simulink model "StateMachine_v3"  (R2015a)
settings: Solver=ode1  StartTime=0.0  StopTime=Inf  FixedStep=0.001  RelTol=1e-3
PreLoadFcn:
  | LoadVar
PostLoadFcn:
  | , if any(exist('dsrtsu_mdlpostloadfcn', 'file') == [2, 3, 6]), try dsrtsu_mdlpostloadfcn('Execute', bdroot); catch fprintf('Error in PostLoadFcn (dsrtsu_mdlpostloadfcn) for model "%s":\n %s\n', bdroot, lasterr); end, end,
values from neighbouring files (symbols this model uses):
  AllowReset = 0    [LoadVar.m]
  Brake_Limits = [Brake_lowerlim1,Brake_upperlim1,Brake_lowerlim2,Brake_upperlim2]    [LoadVar.m]
  DcCLimGen = 0    [LoadVar.m]
  DcCLimMot = 20    [LoadVar.m]
  DcVLimGen = 400    [LoadVar.m]
  DcVLimMot = 280    [LoadVar.m]
  DifferentialFactor = 0.5    [LoadVar.m]
  MaxDisplacementSteeringRack = 21.08    [LoadVar.m]
  MaxSteeringAngle = 24.635    [LoadVar.m]
  MechPwrMaxGen = 3000    [LoadVar.m]
  MechPwrMaxMot = 3000    [LoadVar.m]
  PowerLim_W = 3000    [LoadVar.m]
  SpdSlewrate = 1000    [LoadVar.m]
  Steer_Limits = [Steer_lowerlim,Steer_upperlim,Steer_zero]    [LoadVar.m]
  Susp_Limits = [Susp_lowerlim1,Susp_upperlim1,Susp_lowerlim2,Susp_upperlim2,Susp_lowerlim3,Susp_upperlim3,Susp_lowerlim4,Susp_upperlim4]    [LoadVar.m]
  Throttle_Limits = [Throttle_lowerlim1,Throttle_upperlim1,Throttle_lowerlim2,Throttle_upperlim2]    [LoadVar.m]
  TrqSlewrate = 3    [LoadVar.m]
libraries: rtican x25, rti1401lib_adc_type4 x16, rti1401lib_dio_type3 x16, rtilib1401 x1
(part 3 of 7)

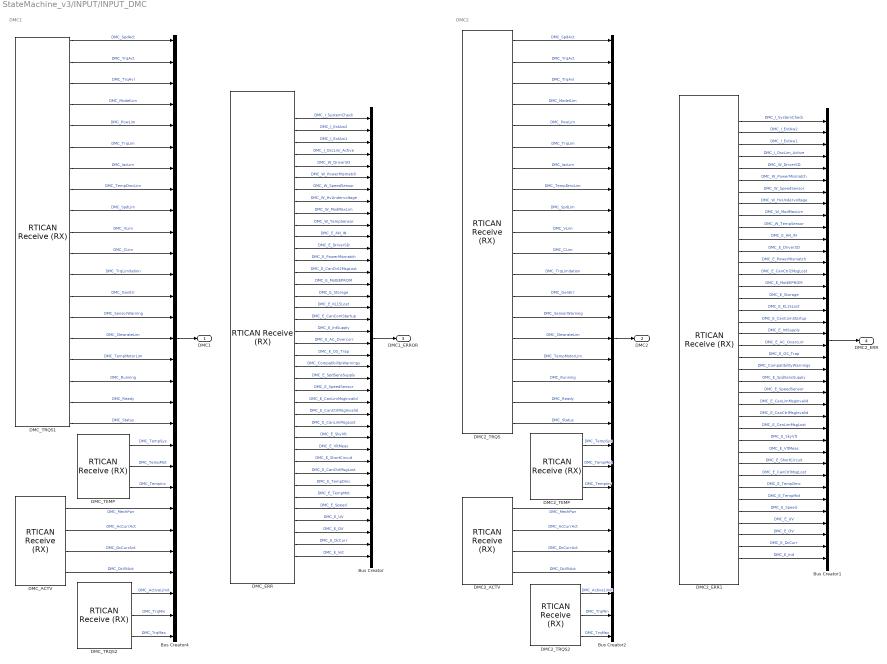
== system StateMachine_v3/INPUT/INPUT_DMC ==
  note: DMC2
  note: DMC1
  Bus Creator : BusCreator  Inputs=38
  Bus Creator1 : BusCreator  Inputs=38
  Bus Creator2 : BusCreator  Inputs=29
  Bus Creator4 : BusCreator  Inputs=29
  DMC2_ACTV : rtican/RTICAN Receive (RX)   Reserved1=[]  Reserved2=[]  Reserved3=[]  Reserved4=[]  SfcnMessage=[]  Msg_Struct=[]  BoardTypeNo=[]  BoardNo=[]  ChannelNo=[]  Parameters=[]  DialogFcn=[]  UnitName=[]  Revision=[]  UnitValues=[]  DSProperties=struct('RTI',struct('Version',uint32(5),'BlockType',struct('isSLSource',uint8(1),'isSLSink',uint8(1),'isHWSource',uint8(0),'isHWSink',uint8(0),'isSetup',uint8(0),'isInline',uint8(1),'isNonInline',uint8(0),'isInterrupt',uint8(0),'isChannelwise',uint8(0)),'IOBoardType','RTICAN','UnitType','MESSAGE','Identifier','RX','DialogType','MSVC','BlockSet','RTICAN','SlaveProcessor','CAN'))  RTIBlockInterface=struct('OutputPortsWidth',int32([1 1 1 1]),'OutputPortsActive',[1 1 1 1],'OutputPortsName',{{'DMC_MechPwr','DMC_AcCurrAct','DMC_DcCurrAct','DMC_DcVltAct'}},'OutputPortsDataType',{{'SS_DOUBLE','SS_DOUBLE','SS_DOUBLE','SS_DOUBLE'}},'OutputPortsLabel',{{'DMC_MechPwr','DMC_AcCurrAct','DMC_DcCurrAct','DMC_DcVltAct'}},'OutputPortsLabelMode','ON','InputPortsWidth',int32(0),'InputPortsActive',0,'DialogFcn','rtican_message_interface_gui','BlockDisplay',{{'','center'}},'IconTransparency','on','ParameterTunableNames',{{}},'InitLevel',3,'BlockName',struct('Token',{{'DMC2_ACTV'}}),'SampleTime',{{-1}},'TriggerPort',{{'none'}},'EnablePort',{{'none'}})  RTIBlockParameters=struct('BoardTypeNo',{{1,'OFF',[]}},'BoardNo',{{2,'ON',[1 16]}},'ChannelNo',{{1,'ON',[1 2]}},'Parameters',{{struct('DataFileSupport',struct('DataFileSelectedMaster',1,'DataFileSelectedLocal',0,'DataFileName','c:\users\powertrain_software\desktop\brusa_02-01-02_rev02-2\documentation\dmc5_can_spec_3.9.dbc|','DataFileDate',{{{['14-dec-2011 16:00:26']}}},'SelectedFile',['<no file selected>']),'Options',struct('StatusSelected',0,'TimeSelected',0,'DeltaTimeSelected',0,'BytePortSelected',0,'MessageLengthSelected',0,'TriggerPort',struct('Selected',0,'TriggerType',0),'UserCoding',struct('Selected',0,'InterfaceFile','UserDecodingFile','FcnName','UserDecodeFcn','InportSelected',0,'InportWidth',1,'OutportSelected',0,'OutportWidth',1),'EnablePortSelected',0,'SignalOnPortnameSelected',1,'UseRXService',0),'Message',struct('MsgOnBlocknameSelected',1,'MsgName','DMC2_ACTV','MsgIdFormat',0,'MsgId',604,'MsgLength',8,'NumSignals',4,'SampleTime',-1,'Signal',struct('SgnName',{'DMC_MechPwr','DMC_AcCurrAct','DMC_DcCurrAct','DMC_DcVltAct'},'SgnStartBit',{0,16,32,48},'SgnLength',{16,16,16,16},'SgnType',{0,0,0,0},'ModeValue',{-1,-1,-1,-1},'DataType',{1,0,1,0},'ByteLayout',{2,2,2,2},'Factor',{16,0.25,0.1,0.1},'Offset',{0,0,0,0},'SgnComment',{{['DMC_MechPwr has new scaling compared to older DMC5 SW Versions!']},{['actual AC current peak value']},{['actual dc current']},{['actual dc voltage']}},'SgnUnit',{'W','A','A','V'},'Min',{-524288,0,-3276.8,0},'Max',{524272,16383.75,3276.7,6553.5},'SLDataType',{'SS_DOUBLE','SS_DOUBLE','SS_DOUBLE','SS_DOUBLE'}),'MsgIdNumFormat',1,'MsgComment',{{''}}),'Version',1.2,'general',struct('isFromLib',0)),'OFF',[]}},'GroupId',{{struct('Group',{{'RTICAN'}},'No',3,'Behavior',{{'NAMECHANGE'}},'BlockType',{{'SINK'}},'NameChangeFlag',0),'OFF',[]}},'SFcnRTICANMessage',{{struct('MsgType','RX','SFcnPortType','Scalar','MsgName','DMC2_ACTV','MsgIdFormat','STD','MsgId',604,'MsgLength',8,'NumSignals',4,'SampleTime',-1,'Signal',struct('SgnName',{'DMC_MechPwr','DMC_AcCurrAct','DMC_DcCurrAct','DMC_DcVltAct'},'SgnStartBit',{0,16,32,48},'SgnLength',{16,16,16,16},'SgnType',{'standard','standard','standard','standard'},'ModeValue',{-1,-1,-1,-1},'DataType',{['signed int'],['unsigned int'],['signed int'],['unsigned int']},'ByteLayout',{['motorola back.'],['motorola back.'],['motorola back.'],['motorola back.']},'Factor',{16,0.25,0.1,0.1},'Offset',{0,0,0,0},'SLDataType',{'SS_DOUBLE','SS_DOUBLE','SS_DOUBLE','SS_DOUBLE'}),'StatusSelected','no','TimeSelected','no','DeltaTimeSelected','no','BytePortSelected','no','MessageLengthSelected','no','TriggerPort',struct('Selected','no','TriggerType',0),'UserCoding',struct('Selected','no','InterfaceFile','UserDecodingFile','FcnName','UserDecodeFcn','InportSelected','no','InportWidth',1,'OutportSelected','no','OutportWidth',1),'EnablePortSelected','no','UseRXService','no','BoardType','DS1','BoardNo',2,'ControllerNo',1),'OFF',[]}},'TLCFileName',{{'rtican_rx_message','OFF',[]}})  RTISFcnParameters=struct('SFcnRTICANMessage','struct','TLCFileName','char')  RTIBlockParaDefault=struct('BoardTypeNo',4302,'BoardNo',1,'ChannelNo',1,'Parameters',struct('DataFileSupport',struct('DataFileSelectedMaster',0,'DataFileSelectedLocal',0,'DataFileName','','DataFileDate','','SelectedFile',['<no file selected>']),'Options',struct('StatusSelected',1,'TimeSelected',1,'DeltaTimeSelected',1,'BytePortSelected',0,'MessageLengthSelected',0,'TriggerPort',struct('Selected',0,'TriggerType','rising'),'UserCoding',struct('Selected',0,'InterfaceFile','UserDecodingFile','FcnName','UserDecodeFcn','InportSelected',0,'InportWidth',1,'OutportSelected',0,'OutportWidth',1),'EnablePortSelected',0,'SignalOnPortnameSelected',1,'UseRXService',0),'Message',struct('MsgOnBlocknameSelected',0,'MsgName',['RX Message'],'MsgIdFormat',0,'MsgId',100,'MsgLength',8,'NumSignals',1,'SampleTime',-1,'Signal',struct('SgnName',['RX signal'],'SgnStartBit',0,'SgnLength',8,'SgnType',0,'ModeValue',-1,'DataType',0,'SLDataType','SS_DOUBLE','ByteLayout',0,'Factor',1,'Offset',0,'Min',0,'Max',255,'SgnComment',{{}},'SgnUnit',''),'MsgIdNumFormat',0,'MsgComment',{{''}}),'Version',1.2,'general',struct('isFromLib',1)),'GroupId',struct('Group',{{'RTICAN'}},'No',1,'Behavior',{{'NAMECHANGE'}},'BlockType',{{'SINK'}},'NameChangeFlag',0),'SFcnRTICANMessage',struct('MsgType','RX','MsgName',['RX Message'],'MsgIdFormat','STD','MsgId',100,'MsgLength',8,'NumSignals',1,'SampleTime',-1,'Signal',struct('SgnName',['RX signal'],'SgnStartBit',0,'SgnLength',8,'SgnType','standard','ModeValue',-1,'DataType',['unsigned int'],'ByteLayout',['little endian'],'SLDataType','SS_DOUBLE','Factor',1,'Offset',0),'StatusSelected','yes','TimeSelected','yes','DeltaTimeSelected','yes','BytePortSelected','no','MessageLengthSelected','no','EnablePortSelected','no','UserCoding',struct('Selected','no','InterfaceFile','UserDecodingFile','FcnName','UserDecodeFcn','InportSelected','no','InportWidth',1,'OutportSelected','no','OutportWidth',1),'TriggerPort',struct('Selected','no','TriggerType','rising'),'UseRXService','no','BoardType','DS4302','BoardNo',1,'ControllerNo',1,'SFcnPortType','Scalar'),'TLCFileName','rtican_rx_message')
      settings: AttributesFormatString=Group Id: RTICAN3\n
  DMC2_ERR1 : rtican/RTICAN Receive (RX)   Reserved1=[]  Reserved2=[]  Reserved3=[]  Reserved4=[]  SfcnMessage=[]  Msg_Struct=[]  BoardTypeNo=[]  BoardNo=[]  ChannelNo=[]  Parameters=[]  DialogFcn=[]  UnitName=[]  Revision=[]  UnitValues=[]  DSProperties=struct('RTI',struct('Version',uint32(5),'BlockType',struct('isSLSource',uint8(1),'isSLSink',uint8(1),'isHWSource',uint8(0),'isHWSink',uint8(0),'isSetup',uint8(0),'isInline',uint8(1),'isNonInline',uint8(0),'isInterrupt',uint8(0),'isChannelwise',uint8(0)),'IOBoardType','RTICAN','UnitType','MESSAGE','Identifier','RX','DialogType','MSVC','BlockSet','RTICAN','SlaveProcessor','CAN'))  RTIBlockInterface=struct('OutputPortsWidth',int32([1 1 1 1 1 1 1 1 1 1 1 1 1 1 1 1 1 1 1 1 1 1 1 1 1 1 1 1 1 1 1 1 1 1 1 1 1 1]),'OutputPortsActive',[1 1 1 1 1 1 1 1 1 1 1 1 1 1 1 1 1 1 1 1 1 1 1 1 1 1 1 1 1 1 1 1 1 1 1 1 1 1],'OutputPortsName',{{'DMC_I_SystemCheck','DMC_I_ExtAw2','DMC_I_ExtAw1','DMC_I_OscLim_Active','DMC_W_DriverSD','DMC_W_PowerMismatch','DMC_W_SpeedSensor','DMC_W_HvUndervoltage','DMC_W_ModMaxLim','DMC_W_TempSensor','DMC_E_AN_IN','DMC_E_DriverSD','DMC_E_PowerMismatch','DMC_E_CanCtrl2MsgLost','DMC_E_MotEEPROM','DMC_E_Storage','DMC_E_KL15Lost','DMC_E_CanComStartup','DMC_E_IntSupply','DMC_E_AC_Overcurr','DMC_E_OS_Trap','DMC_CompatibilityWarnings','DMC_E_SpdSensSupply','DMC_E_SpeedSensor','DMC_E_CanLimMsgInvalid','DMC_E_CanCtrlMsgInvalid','DMC_E_CanLimMsgLost','DMC_E_SkyVlt','DMC_E_VltMeas','DMC_E_ShortCircuit','DMC_E_CanCtrlMsgLost','DMC_E_TempDmc','DMC_E_TempMot','DMC_E_Speed','DMC_E_UV','DMC_E_OV','DMC_E_DcCurr','DMC_E_Init'}},'OutputPortsDataType',{{'SS_DOUBLE','SS_DOUBLE','SS_DOUBLE','SS_DOUBLE','SS_DOUBLE','SS_DOUBLE','SS_DOUBLE','SS_DOUBLE','SS_DOUBLE','SS_DOUBLE','SS_DOUBLE','SS_DOUBLE','SS_DOUBLE','SS_DOUBLE','SS_DOUBLE','SS_DOUBLE','SS_DOUBLE','SS_DOUBLE','SS_DOUBLE','SS_DOUBLE','SS_DOUBLE','SS_DOUBLE','SS_DOUBLE','SS_DOUBLE','SS_DOUBLE','SS_DOUBLE','SS_DOUBLE','SS_DOUBLE','SS_DOUBLE','SS_DOUBLE','SS_DOUBLE','SS_DOUBLE','SS_DOUBLE','SS_DOUBLE','SS_DOUBLE','SS_DOUBLE','SS_DOUBLE','SS_DOUBLE'}},'OutputPortsLabel',{{'DMC_I_SystemCheck','DMC_I_ExtAw2','DMC_I_ExtAw1','DMC_I_OscLim_Active','DMC_W_DriverSD','DMC_W_PowerMismatch','DMC_W_SpeedSensor','DMC_W_HvUndervoltage','DMC_W_ModMaxLim','DMC_W_TempSensor','DMC_E_AN_IN','DMC_E_DriverSD','DMC_E_PowerMismatch','DMC_E_CanCtrl2MsgLost','DMC_E_MotEEPROM','DMC_E_Storage','DMC_E_KL15Lost','DMC_E_CanComStartup','DMC_E_IntSupply','DMC_E_AC_Overcurr','DMC_E_OS_Trap','DMC_CompatibilityWarnings','DMC_E_SpdSensSupply','DMC_E_SpeedSensor','DMC_E_CanLimMsgInvalid','DMC_E_CanCtrlMsgInvalid','DMC_E_CanLimMsgLost','DMC_E_SkyVlt','DMC_E_VltMeas','DMC_E_ShortCircuit','DMC_E_CanCtrlMsgLost','DMC_E_TempDmc','DMC_E_TempMot','DMC_E_Speed','DMC_E_UV','DMC_E_OV','DMC_E_DcCurr','DMC_E_Init'}},'OutputPortsLabelMode','ON','InputPortsWidth',int32(0),'InputPortsActive',0,'DialogFcn','rtican_message_interface_gui','BlockDisplay',{{'','center'}},'IconTransparency','on','ParameterTunableNames',{{}},'InitLevel',3,'BlockName',struct('Token',{{'DMC2_ERR'}}),'SampleTime',{{-1}},'TriggerPort',{{'none'}},'EnablePort',{{'none'}})  RTIBlockParameters=struct('BoardTypeNo',{{1,'OFF',[]}},'BoardNo',{{2,'ON',[1 16]}},'ChannelNo',{{1,'ON',[1 2]}},'Parameters',{{struct('DataFileSupport',struct('DataFileSelectedMaster',1,'DataFileSelectedLocal',0,'DataFileName','c:\users\powertrain_software\desktop\brusa_02-01-02_rev02-2\documentation\dmc5_can_spec_3.9.dbc|','DataFileDate',{{{['14-dec-2011 16:00:26']}}},'SelectedFile',['<no file selected>']),'Options',struct('StatusSelected',0,'TimeSelected',0,'DeltaTimeSelected',0,'BytePortSelected',0,'MessageLengthSelected',0,'TriggerPort',struct('Selected',0,'TriggerType',0),'UserCoding',struct('Selected',0,'InterfaceFile','UserDecodingFile','FcnName','UserDecodeFcn','InportSelected',0,'InportWidth',1,'OutportSelected',0,'OutportWidth',1),'EnablePortSelected',0,'SignalOnPortnameSelected',1,'UseRXService',0),'Message',struct('MsgOnBlocknameSelected',1,'MsgName','DMC2_ERR','MsgIdFormat',0,'MsgId',605,'MsgLength',8,'NumSignals',38,'SampleTime',-1,'Signal',struct('SgnName',{'DMC_I_SystemCheck','DMC_I_ExtAw2','DMC_I_ExtAw1','DMC_I_OscLim_Active','DMC_W_DriverSD','DMC_W_PowerMismatch','DMC_W_SpeedSensor','DMC_W_HvUndervoltage','DMC_W_ModMaxLim','DMC_W_TempSensor','DMC_E_AN_IN','DMC_E_DriverSD','DMC_E_PowerMismatch','DMC_E_CanCtrl2MsgLost','DMC_E_MotEEPROM','DMC_E_Storage','DMC_E_KL15Lost','DMC_E_CanComStartup','DMC_E_IntSupply','DMC_E_AC_Overcurr','DMC_E_OS_Trap','DMC_CompatibilityWarnings','DMC_E_SpdSensSupply','DMC_E_SpeedSensor','DMC_E_CanLimMsgInvalid','DMC_E_CanCtrlMsgInvalid','DMC_E_CanLimMsgLost','DMC_E_SkyVlt','DMC_E_VltMeas','DMC_E_ShortCircuit','DMC_E_CanCtrlMsgLost','DMC_E_TempDmc','DMC_E_TempMot','DMC_E_Speed','DMC_E_UV','DMC_E_OV','DMC_E_DcCurr','DMC_E_Init'},'SgnStartBit',{0,1,2,3,10,11,12,13,14,15,16,22,23,24,25,26,27,28,29,30,31,32,48,49,50,51,52,53,54,55,56,57,58,59,60,61,62,63},'SgnLength',{1,1,1,1,1,1,1,1,1,1,1,1,1,1,1,1,1,1,1,1,1,16,1,1,1,1,1,1,1,1,1,1,1,1,1,1,1,1},'SgnType',{0,0,0,0,0,0,0,0,0,0,0,0,0,0,0,0,0,0,0,0,0,0,0,0,0,0,0,0,0,0,0,0,0,0,0,0,0,0},'ModeValue',{-1,-1,-1,-1,-1,-1,-1,-1,-1,-1,-1,-1,-1,-1,-1,-1,-1,-1,-1,-1,-1,-1,-1,-1,-1,-1,-1,-1,-1,-1,-1,-1,-1,-1,-1,-1,-1,-1},'DataType',{0,0,0,0,0,0,0,0,0,0,0,0,0,0,0,0,0,0,0,0,0,0,0,0,0,0,0,0,0,0,0,0,0,0,0,0,0,0},'ByteLayout',{2,2,2,2,2,2,2,2,2,2,2,2,2,2,2,2,2,2,2,2,2,2,2,2,2,2,2,2,2,2,2,2,2,2,2,2,2,2},'Factor',{1,1,1,1,1,1,1,1,1,1,1,1,1,1,1,1,1,1,1,1,1,1,1,1,1,1,1,1,1,1,1,1,1,1,1,1,1,1},'Offset',{0,0,0,0,0,0,0,0,0,0,0,0,0,0,0,0,0,0,0,0,0,0,0,0,0,0,0,0,0,0,0,0,0,0,0,0,0,0},'SgnComment',{{['warnings are described in seperate document']},{['warnings are described in seperate document']},{['warnings are described in seperate document']},{['warnings are described in seperate document']},{['errors are described in seperate document']},{['warnings are described in seperate document']},{['warnings are described in seperate document']},{['warnings are described in seperate document']},{['warnings are described in seperate document']},{['warnings are described in seperate document']},{['errors are described in seperate document']},{['errors are described in seperate document']},{['errors are described in seperate document']},{['errors are described in seperate document']},{['errors are described in seperate document']},{['errors are described in seperate document']},{['errors are described in seperate document']},{['errors are described in seperate document']},{['errors are described in seperate document']},{['errors are described in seperate document']},{['errors are described in seperate document']},{['Warning Bitmap CAN Matrix <= 3.6 is sent at this Position']},{['errors are described in seperate document']},{['errors are described in seperate document']},{['errors are described in seperate document']},{['errors are described in seperate document']},{['errors are described in seperate document']},{['errors are described in seperate document']},{['errors are described in seperate document']},{['errors are described in seperate document']},{['errors are described in seperate document']},{['errors are described in seperate document']},{['errors are described in seperate document']},{['errors are described in seperate document']},{['errors are described in seperate document']},{['errors are described in seperate document']},{['errors are described in seperate document']},{['errors are described in seperate document']}},'SgnUnit',{'','','','','','','','','','','','','','','','','','','','','','','','','','','','','','','','','','','','','',''},'Min',{0,0,0,0,0,0,0,0,0,0,0,0,0,0,0,0,0,0,0,0,0,0,0,0,0,0,0,0,0,0,0,0,0,0,0,0,0,0},'Max',{0,0,0,0,0,0,0,0,0,0,0,0,0,0,0,0,0,0,0,0,0,0,0,0,0,0,0,0,0,0,0,0,0,0,0,0,0,0},'SLDataType',{'SS_DOUBLE','SS_DOUBLE','SS_DOUBLE','SS_DOUBLE','SS_DOUBLE','SS_DOUBLE','SS_DOUBLE','SS_DOUBLE','SS_DOUBLE','SS_DOUBLE','SS_DOUBLE','SS_DOUBLE','SS_DOUBLE','SS_DOUBLE','SS_DOUBLE','SS_DOUBLE','SS_DOUBLE','SS_DOUBLE','SS_DOUBLE','SS_DOUBLE','SS_DOUBLE','SS_DOUBLE','SS_DOUBLE','SS_DOUBLE','SS_DOUBLE','SS_DOUBLE','SS_DOUBLE','SS_DOUBLE','SS_DOUBLE','SS_DOUBLE','SS_DOUBLE','SS_DOUBLE','SS_DOUBLE','SS_DOUBLE','SS_DOUBLE','SS_DOUBLE','SS_DOUBLE','SS_DOUBLE'}),'MsgIdNumFormat',1,'MsgComment',{{''}}),'Version',1.2,'general',struct('isFromLib',0)),'OFF',[]}},'GroupId',{{struct('Group',{{'RTICAN'}},'No',3,'Behavior',{{'NAMECHANGE'}},'BlockType',{{'SINK'}},'NameChangeFlag',0),'OFF',[]}},'SFcnRTICANMessage',{{struct('MsgType','RX','SFcnPortType','Scalar','MsgName','DMC2_ERR','MsgIdFormat','STD','MsgId',605,'MsgLength',8,'NumSignals',38,'SampleTime',-1,'Signal',struct('SgnName',{'DMC_I_SystemCheck','DMC_I_ExtAw2','DMC_I_ExtAw1','DMC_I_OscLim_Active','DMC_W_DriverSD','DMC_W_PowerMismatch','DMC_W_SpeedSensor','DMC_W_HvUndervoltage','DMC_W_ModMaxLim','DMC_W_TempSensor','DMC_E_AN_IN','DMC_E_DriverSD','DMC_E_PowerMismatch','DMC_E_CanCtrl2MsgLost','DMC_E_MotEEPROM','DMC_E_Storage','DMC_E_KL15Lost','DMC_E_CanComStartup','DMC_E_IntSupply','DMC_E_AC_Overcurr','DMC_E_OS_Trap','DMC_CompatibilityWarnings','DMC_E_SpdSensSupply','DMC_E_SpeedSensor','DMC_E_CanLimMsgInvalid','DMC_E_CanCtrlMsgInvalid','DMC_E_CanLimMsgLost','DMC_E_SkyVlt','DMC_E_VltMeas','DMC_E_ShortCircuit','DMC_E_CanCtrlMsgLost','DMC_E_TempDmc','DMC_E_TempMot','DMC_E_Speed','DMC_E_UV','DMC_E_OV','DMC_E_DcCurr','DMC_E_Init'},'SgnStartBit',{0,1,2,3,10,11,12,13,14,15,16,22,23,24,25,26,27,28,29,30,31,32,48,49,50,51,52,53,54,55,56,57,58,59,60,61,62,63},'SgnLength',{1,1,1,1,1,1,1,1,1,1,1,1,1,1,1,1,1,1,1,1,1,16,1,1,1,1,1,1,1,1,1,1,1,1,1,1,1,1},'SgnType',{'standard','standard','standard','standard','standard','standard','standard','standard','standard','standard','standard','standard','standard','standard','standard','standard','standard','standard','standard','standard','standard','standard','standard','standard','standard','standard','standard','standard','standard','standard','standard','standard','standard','standard','standard','standard','standard','standard'},'ModeValue',{-1,-1,-1,-1,-1,-1,-1,-1,-1,-1,-1,-1,-1,-1,-1,-1,-1,-1,-1,-1,-1,-1,-1,-1,-1,-1,-1,-1,-1,-1,-1,-1,-1,-1,-1,-1,-1,-1},'DataType',{['unsigned int'],['unsigned int'],['unsigned int'],['unsigned int'],['unsigned int'],['unsigned int'],['unsigned int'],['unsigned int'],['unsigned int'],['unsigned int'],['unsigned int'],['unsigned int'],['unsigned int'],['unsigned int'],['unsigned int'],['unsigned int'],['unsigned int'],['unsigned int'],['unsigned int'],['unsigned int'],['unsigned int'],['unsigned int'],['unsigned int'],['unsigned int'],['unsigned int'],['unsigned int'],['unsigned int'],['unsigned int'],['unsigned int'],['unsigned int'],['unsigned int'],['unsigned int'],['unsigned int'],['unsigned int'],['unsigned int'],['unsigned int'],['unsigned int'],['unsigned int']},'ByteLayout',{['motorola back.'],['motorola back.'],['motorola back.'],['motorola back.'],['motorola back.'],['motorola back.'],['motorola back.'],['motorola back.'],['motorola back.'],['motorola back.'],['motorola back.'],['motorola back.'],['motorola back.'],['motorola back.'],['motorola back.'],['motorola back.'],['motorola back.'],['motorola back.'],['motorola back.'],['motorola back.'],['motorola back.'],['motorola back.'],['motorola back.'],['motorola back.'],['motorola back.'],['motorola back.'],['motorola back.'],['motorola back.'],['motorola back.'],['motorola back.'],['motorola back.'],['motorola back.'],['motorola back.'],['motorola back.'],['motorola back.'],['motorola back.'],['motorola back.'],['motorola back.']},'Factor',{1,1,1,1,1,1,1,1,1,1,1,1,1,1,1,1,1,1,1,1,1,1,1,1,1,1,1,1,1,1,1,1,1,1,1,1,1,1},'Offset',{0,0,0,0,0,0,0,0,0,0,0,0,0,0,0,0,0,0,0,0,0,0,0,0,0,0,0,0,0,0,0,0,0,0,0,0,0,0},'SLDataType',{'SS_DOUBLE','SS_DOUBLE','SS_DOUBLE','SS_DOUBLE','SS_DOUBLE','SS_DOUBLE','SS_DOUBLE','SS_DOUBLE','SS_DOUBLE','SS_DOUBLE','SS_DOUBLE','SS_DOUBLE','SS_DOUBLE','SS_DOUBLE','SS_DOUBLE','SS_DOUBLE','SS_DOUBLE','SS_DOUBLE','SS_DOUBLE','SS_DOUBLE','SS_DOUBLE','SS_DOUBLE','SS_DOUBLE','SS_DOUBLE','SS_DOUBLE','SS_DOUBLE','SS_DOUBLE','SS_DOUBLE','SS_DOUBLE','SS_DOUBLE','SS_DOUBLE','SS_DOUBLE','SS_DOUBLE','SS_DOUBLE','SS_DOUBLE','SS_DOUBLE','SS_DOUBLE','SS_DOUBLE'}),'StatusSelected','no','TimeSelected','no','DeltaTimeSelected','no','BytePortSelected','no','MessageLengthSelected','no','TriggerPort',struct('Selected','no','TriggerType',0),'UserCoding',struct('Selected','no','InterfaceFile','UserDecodingFile','FcnName','UserDecodeFcn','InportSelected','no','InportWidth',1,'OutportSelected','no','OutportWidth',1),'EnablePortSelected','no','UseRXService','no','BoardType','DS1','BoardNo',2,'ControllerNo',1),'OFF',[]}},'TLCFileName',{{'rtican_rx_message','OFF',[]}})  RTISFcnParameters=struct('SFcnRTICANMessage','struct','TLCFileName','char')  RTIBlockParaDefault=struct('BoardTypeNo',4302,'BoardNo',1,'ChannelNo',1,'Parameters',struct('DataFileSupport',struct('DataFileSelectedMaster',0,'DataFileSelectedLocal',0,'DataFileName','','DataFileDate','','SelectedFile',['<no file selected>']),'Options',struct('StatusSelected',1,'TimeSelected',1,'DeltaTimeSelected',1,'BytePortSelected',0,'MessageLengthSelected',0,'TriggerPort',struct('Selected',0,'TriggerType','rising'),'UserCoding',struct('Selected',0,'InterfaceFile','UserDecodingFile','FcnName','UserDecodeFcn','InportSelected',0,'InportWidth',1,'OutportSelected',0,'OutportWidth',1),'EnablePortSelected',0,'SignalOnPortnameSelected',1,'UseRXService',0),'Message',struct('MsgOnBlocknameSelected',0,'MsgName',['RX Message'],'MsgIdFormat',0,'MsgId',100,'MsgLength',8,'NumSignals',1,'SampleTime',-1,'Signal',struct('SgnName',['RX signal'],'SgnStartBit',0,'SgnLength',8,'SgnType',0,'ModeValue',-1,'DataType',0,'SLDataType','SS_DOUBLE','ByteLayout',0,'Factor',1,'Offset',0,'Min',0,'Max',255,'SgnComment',{{}},'SgnUnit',''),'MsgIdNumFormat',0,'MsgComment',{{''}}),'Version',1.2,'general',struct('isFromLib',1)),'GroupId',struct('Group',{{'RTICAN'}},'No',1,'Behavior',{{'NAMECHANGE'}},'BlockType',{{'SINK'}},'NameChangeFlag',0),'SFcnRTICANMessage',struct('MsgType','RX','MsgName',['RX Message'],'MsgIdFormat','STD','MsgId',100,'MsgLength',8,'NumSignals',1,'SampleTime',-1,'Signal',struct('SgnName',['RX signal'],'SgnStartBit',0,'SgnLength',8,'SgnType','standard','ModeValue',-1,'DataType',['unsigned int'],'ByteLayout',['little endian'],'SLDataType','SS_DOUBLE','Factor',1,'Offset',0),'StatusSelected','yes','TimeSelected','yes','DeltaTimeSelected','yes','BytePortSelected','no','MessageLengthSelected','no','EnablePortSelected','no','UserCoding',struct('Selected','no','InterfaceFile','UserDecodingFile','FcnName','UserDecodeFcn','InportSelected','no','InportWidth',1,'OutportSelected','no','OutportWidth',1),'TriggerPort',struct('Selected','no','TriggerType','rising'),'UseRXService','no','BoardType','DS4302','BoardNo',1,'ControllerNo',1,'SFcnPortType','Scalar'),'TLCFileName','rtican_rx_message')
      settings: AttributesFormatString=Group Id: RTICAN3\n
  DMC2_TEMP : rtican/RTICAN Receive (RX)   Reserved1=[]  Reserved2=[]  Reserved3=[]  Reserved4=[]  SfcnMessage=[]  Msg_Struct=[]  BoardTypeNo=[]  BoardNo=[]  ChannelNo=[]  Parameters=[]  DialogFcn=[]  UnitName=[]  Revision=[]  UnitValues=[]  DSProperties=struct('RTI',struct('Version',uint32(5),'BlockType',struct('isSLSource',uint8(1),'isSLSink',uint8(1),'isHWSource',uint8(0),'isHWSink',uint8(0),'isSetup',uint8(0),'isInline',uint8(1),'isNonInline',uint8(0),'isInterrupt',uint8(0),'isChannelwise',uint8(0)),'IOBoardType','RTICAN','UnitType','MESSAGE','Identifier','RX','DialogType','MSVC','BlockSet','RTICAN','SlaveProcessor','CAN'))  RTIBlockInterface=struct('OutputPortsWidth',int32([1 1 1]),'OutputPortsActive',[1 1 1],'OutputPortsName',{{'DMC_TempSys','DMC_TempMot','DMC_TempInv'}},'OutputPortsDataType',{{'SS_DOUBLE','SS_DOUBLE','SS_DOUBLE'}},'OutputPortsLabel',{{'DMC_TempSys','DMC_TempMot','DMC_TempInv'}},'OutputPortsLabelMode','ON','InputPortsWidth',int32(0),'InputPortsActive',0,'DialogFcn','rtican_message_interface_gui','BlockDisplay',{{'','center'}},'IconTransparency','on','ParameterTunableNames',{{}},'InitLevel',3,'BlockName',struct('Token',{{'DMC2_TEMP'}}),'SampleTime',{{-1}},'TriggerPort',{{'none'}},'EnablePort',{{'none'}})  RTIBlockParameters=struct('BoardTypeNo',{{1,'OFF',[]}},'BoardNo',{{2,'ON',[1 16]}},'ChannelNo',{{1,'ON',[1 2]}},'Parameters',{{struct('DataFileSupport',struct('DataFileSelectedMaster',1,'DataFileSelectedLocal',0,'DataFileName','c:\users\powertrain_software\desktop\brusa_02-01-02_rev02-2\documentation\dmc5_can_spec_3.9.dbc|','DataFileDate',{{{['14-dec-2011 16:00:26']}}},'SelectedFile',['<no file selected>']),'Options',struct('StatusSelected',0,'TimeSelected',0,'DeltaTimeSelected',0,'BytePortSelected',0,'MessageLengthSelected',0,'TriggerPort',struct('Selected',0,'TriggerType',0),'UserCoding',struct('Selected',0,'InterfaceFile','UserDecodingFile','FcnName','UserDecodeFcn','InportSelected',0,'InportWidth',1,'OutportSelected',0,'OutportWidth',1),'EnablePortSelected',0,'SignalOnPortnameSelected',1,'UseRXService',0),'Message',struct('MsgOnBlocknameSelected',1,'MsgName','DMC2_TEMP','MsgIdFormat',0,'MsgId',1113,'MsgLength',8,'NumSignals',3,'SampleTime',-1,'Signal',struct('SgnName',{'DMC_TempSys','DMC_TempMot','DMC_TempInv'},'SgnStartBit',{24,32,48},'SgnLength',{8,16,16},'SgnType',{0,0,0},'ModeValue',{-1,-1,-1},'DataType',{0,1,1},'ByteLayout',{2,2,2},'Factor',{1,0.5,0.5},'Offset',{-50,0,0},'SgnComment',{{['temperature dmc (inverter)']},{['temperature motor']},{['temperature dmc (inverter)']}},'SgnUnit',{'°C','°C','°C'},'Min',{-50,-16384,-16384},'Max',{205,16383.5,16383.5},'SLDataType',{'SS_DOUBLE','SS_DOUBLE','SS_DOUBLE'}),'MsgIdNumFormat',1,'MsgComment',{{''}}),'Version',1.2,'general',struct('isFromLib',0)),'OFF',[]}},'GroupId',{{struct('Group',{{'RTICAN'}},'No',3,'Behavior',{{'NAMECHANGE'}},'BlockType',{{'SINK'}},'NameChangeFlag',0),'OFF',[]}},'SFcnRTICANMessage',{{struct('MsgType','RX','SFcnPortType','Scalar','MsgName','DMC2_TEMP','MsgIdFormat','STD','MsgId',1113,'MsgLength',8,'NumSignals',3,'SampleTime',-1,'Signal',struct('SgnName',{'DMC_TempSys','DMC_TempMot','DMC_TempInv'},'SgnStartBit',{24,32,48},'SgnLength',{8,16,16},'SgnType',{'standard','standard','standard'},'ModeValue',{-1,-1,-1},'DataType',{['unsigned int'],['signed int'],['signed int']},'ByteLayout',{['motorola back.'],['motorola back.'],['motorola back.']},'Factor',{1,0.5,0.5},'Offset',{-50,0,0},'SLDataType',{'SS_DOUBLE','SS_DOUBLE','SS_DOUBLE'}),'StatusSelected','no','TimeSelected','no','DeltaTimeSelected','no','BytePortSelected','no','MessageLengthSelected','no','TriggerPort',struct('Selected','no','TriggerType',0),'UserCoding',struct('Selected','no','InterfaceFile','UserDecodingFile','FcnName','UserDecodeFcn','InportSelected','no','InportWidth',1,'OutportSelected','no','OutportWidth',1),'EnablePortSelected','no','UseRXService','no','BoardType','DS1','BoardNo',2,'ControllerNo',1),'OFF',[]}},'TLCFileName',{{'rtican_rx_message','OFF',[]}})  RTISFcnParameters=struct('SFcnRTICANMessage','struct','TLCFileName','char')  RTIBlockParaDefault=struct('BoardTypeNo',4302,'BoardNo',1,'ChannelNo',1,'Parameters',struct('DataFileSupport',struct('DataFileSelectedMaster',0,'DataFileSelectedLocal',0,'DataFileName','','DataFileDate','','SelectedFile',['<no file selected>']),'Options',struct('StatusSelected',1,'TimeSelected',1,'DeltaTimeSelected',1,'BytePortSelected',0,'MessageLengthSelected',0,'TriggerPort',struct('Selected',0,'TriggerType','rising'),'UserCoding',struct('Selected',0,'InterfaceFile','UserDecodingFile','FcnName','UserDecodeFcn','InportSelected',0,'InportWidth',1,'OutportSelected',0,'OutportWidth',1),'EnablePortSelected',0,'SignalOnPortnameSelected',1,'UseRXService',0),'Message',struct('MsgOnBlocknameSelected',0,'MsgName',['RX Message'],'MsgIdFormat',0,'MsgId',100,'MsgLength',8,'NumSignals',1,'SampleTime',-1,'Signal',struct('SgnName',['RX signal'],'SgnStartBit',0,'SgnLength',8,'SgnType',0,'ModeValue',-1,'DataType',0,'SLDataType','SS_DOUBLE','ByteLayout',0,'Factor',1,'Offset',0,'Min',0,'Max',255,'SgnComment',{{}},'SgnUnit',''),'MsgIdNumFormat',0,'MsgComment',{{''}}),'Version',1.2,'general',struct('isFromLib',1)),'GroupId',struct('Group',{{'RTICAN'}},'No',1,'Behavior',{{'NAMECHANGE'}},'BlockType',{{'SINK'}},'NameChangeFlag',0),'SFcnRTICANMessage',struct('MsgType','RX','MsgName',['RX Message'],'MsgIdFormat','STD','MsgId',100,'MsgLength',8,'NumSignals',1,'SampleTime',-1,'Signal',struct('SgnName',['RX signal'],'SgnStartBit',0,'SgnLength',8,'SgnType','standard','ModeValue',-1,'DataType',['unsigned int'],'ByteLayout',['little endian'],'SLDataType','SS_DOUBLE','Factor',1,'Offset',0),'StatusSelected','yes','TimeSelected','yes','DeltaTimeSelected','yes','BytePortSelected','no','MessageLengthSelected','no','EnablePortSelected','no','UserCoding',struct('Selected','no','InterfaceFile','UserDecodingFile','FcnName','UserDecodeFcn','InportSelected','no','InportWidth',1,'OutportSelected','no','OutportWidth',1),'TriggerPort',struct('Selected','no','TriggerType','rising'),'UseRXService','no','BoardType','DS4302','BoardNo',1,'ControllerNo',1,'SFcnPortType','Scalar'),'TLCFileName','rtican_rx_message')
      settings: AttributesFormatString=Group Id: RTICAN3\n
  DMC2_TRQS : rtican/RTICAN Receive (RX)   Reserved1=[]  Reserved2=[]  Reserved3=[]  Reserved4=[]  SfcnMessage=[]  Msg_Struct=[]  BoardTypeNo=[]  BoardNo=[]  ChannelNo=[]  Parameters=[]  DialogFcn=[]  UnitName=[]  Revision=[]  UnitValues=[]  DSProperties=struct('RTI',struct('Version',uint32(5),'BlockType',struct('isSLSource',uint8(1),'isSLSink',uint8(1),'isHWSource',uint8(0),'isHWSink',uint8(0),'isSetup',uint8(0),'isInline',uint8(1),'isNonInline',uint8(0),'isInterrupt',uint8(0),'isChannelwise',uint8(0)),'IOBoardType','RTICAN','UnitType','MESSAGE','Identifier','RX','DialogType','MSVC','BlockSet','RTICAN','SlaveProcessor','CAN'))  RTIBlockInterface=struct('OutputPortsWidth',int32([1 1 1 1 1 1 1 1 1 1 1 1 1 1 1 1 1 1 1]),'OutputPortsActive',[1 1 1 1 1 1 1 1 1 1 1 1 1 1 1 1 1 1 1],'OutputPortsName',{{'DMC_SpdAct','DMC_TrqAct','DMC_TrqAvl','DMC_ModelLim','DMC_PowLim','DMC_TrqLim','DMC_IacLim','DMC_TempDmcLim','DMC_SpdLim','DMC_VLim','DMC_CLim','DMC_TrqLimitation','DMC_GenErr','DMC_SensorWarning','DMC_SlewrateLim','DMC_TempMotorLim','DMC_Running','DMC_Ready',['RX status']}},'OutputPortsDataType',{{'SS_DOUBLE','SS_DOUBLE','SS_DOUBLE','SS_DOUBLE','SS_DOUBLE','SS_DOUBLE','SS_DOUBLE','SS_DOUBLE','SS_DOUBLE','SS_DOUBLE','SS_DOUBLE','SS_DOUBLE','SS_DOUBLE','SS_DOUBLE','SS_DOUBLE','SS_DOUBLE','SS_DOUBLE','SS_DOUBLE','SS_DOUBLE'}},'OutputPortsLabel',{{'DMC_SpdAct','DMC_TrqAct','DMC_TrqAvl','DMC_ModelLim','DMC_PowLim','DMC_TrqLim','DMC_IacLim','DMC_TempDmcLim','DMC_SpdLim','DMC_VLim','DMC_CLim','DMC_TrqLimitation','DMC_GenErr','DMC_SensorWarning','DMC_SlewrateLim','DMC_TempMotorLim','DMC_Running','DMC_Ready',''}},'OutputPortsLabelMode','ON','InputPortsWidth',int32(0),'InputPortsActive',0,'DialogFcn','rtican_message_interface_gui','BlockDisplay',{{'','center'}},'IconTransparency','on','ParameterTunableNames',{{}},'InitLevel',3,'BlockName',struct('Token',{{'DMC2_TRQS'}}),'SampleTime',{{-1}},'TriggerPort',{{'none'}},'EnablePort',{{'none'}})  RTIBlockParameters=struct('BoardTypeNo',{{1,'OFF',[]}},'BoardNo',{{2,'ON',[1 16]}},'ChannelNo',{{1,'ON',[1 2]}},'Parameters',{{struct('DataFileSupport',struct('DataFileSelectedMaster',1,'DataFileSelectedLocal',0,'DataFileName','c:\users\powertrain_software\desktop\brusa_02-01-02_rev02-2\documentation\dmc5_can_spec_3.9.dbc|','DataFileDate',{{{['14-dec-2011 16:00:26']}}},'SelectedFile',['<no file selected>']),'Options',struct('StatusSelected',1,'TimeSelected',0,'DeltaTimeSelected',0,'BytePortSelected',0,'MessageLengthSelected',0,'TriggerPort',struct('Selected',0,'TriggerType',0),'UserCoding',struct('Selected',0,'InterfaceFile','UserDecodingFile','FcnName','UserDecodeFcn','InportSelected',0,'InportWidth',1,'OutportSelected',0,'OutportWidth',1),'EnablePortSelected',0,'SignalOnPortnameSelected',1,'UseRXService',0),'Message',struct('MsgOnBlocknameSelected',1,'MsgName','DMC2_TRQS','MsgIdFormat',0,'MsgId',603,'MsgLength',8,'NumSignals',18,'SampleTime',-1,'Signal',struct('SgnName',{'DMC_SpdAct','DMC_TrqAct','DMC_TrqAvl','DMC_ModelLim','DMC_PowLim','DMC_TrqLim','DMC_IacLim','DMC_TempDmcLim','DMC_SpdLim','DMC_VLim','DMC_CLim','DMC_TrqLimitation','DMC_GenErr','DMC_SensorWarning','DMC_SlewrateLim','DMC_TempMotorLim','DMC_Running','DMC_Ready'},'SgnStartBit',{0,16,32,48,49,50,51,52,53,54,55,56,57,58,60,61,62,63},'SgnLength',{16,16,16,1,1,1,1,1,1,1,1,1,1,1,1,1,1,1},'SgnType',{0,0,0,0,0,0,0,0,0,0,0,0,0,0,0,0,0,0},'ModeValue',{-1,-1,-1,-1,-1,-1,-1,-1,-1,-1,-1,-1,-1,-1,-1,-1,-1,-1},'DataType',{1,1,1,0,0,0,0,0,0,0,0,0,0,0,0,0,0,0},'ByteLayout',{2,2,2,2,2,2,2,2,2,2,2,2,2,2,2,2,2,2},'Factor',{1,0.01,0.01,1,1,1,1,1,1,1,1,1,1,1,1,1,1,1},'Offset',{0,0,0,0,0,0,0,0,0,0,0,0,0,0,0,0,0,0},'SgnComment',{{['actual motor speed']},{['actual torque']},{['max available torque']},{['torque limit by motor model']},{['torque limitation by mechanical power']},{['torque limitation by max torque']},{['torque limit by ac current']},{['torque limit by dmc temperature']},{['torque limitation by speed']},{['torque limitation by dc voltage']},{['trq limited by dc current']},{['torque limitation is active']},{['an error bit is set in the error bitmap (DMC_ERR msg)']},{['a warning is set in the warning bitmap (DMC_ERR msg)']},{['torque limitation by max slewrate (torque or speed)']},{['torque limitation by motor temperature']},{['dmc is running']},{['dmc is ready for operation']}},'SgnUnit',{'rpm','Nm','Nm','','','','','','','','','','','','','','',''},'Min',{-32768,-327.68,-327.68,0,0,0,0,0,0,0,0,0,0,0,0,0,0,0},'Max',{23767,327.67,327.67,0,0,0,0,0,0,0,0,0,0,0,0,0,0,0},'SLDataType',{'SS_DOUBLE','SS_DOUBLE','SS_DOUBLE','SS_DOUBLE','SS_DOUBLE','SS_DOUBLE','SS_DOUBLE','SS_DOUBLE','SS_DOUBLE','SS_DOUBLE','SS_DOUBLE','SS_DOUBLE','SS_DOUBLE','SS_DOUBLE','SS_DOUBLE','SS_DOUBLE','SS_DOUBLE','SS_DOUBLE'}),'MsgIdNumFormat',1,'MsgComment',{{''}}),'Version',1.2,'general',struct('isFromLib',0)),'OFF',[]}},'GroupId',{{struct('Group',{{'RTICAN'}},'No',3,'Behavior',{{'NAMECHANGE'}},'BlockType',{{'SINK'}},'NameChangeFlag',0),'OFF',[]}},'SFcnRTICANMessage',{{struct('MsgType','RX','SFcnPortType','Scalar','MsgName','DMC2_TRQS','MsgIdFormat','STD','MsgId',603,'MsgLength',8,'NumSignals',18,'SampleTime',-1,'Signal',struct('SgnName',{'DMC_SpdAct','DMC_TrqAct','DMC_TrqAvl','DMC_ModelLim','DMC_PowLim','DMC_TrqLim','DMC_IacLim','DMC_TempDmcLim','DMC_SpdLim','DMC_VLim','DMC_CLim','DMC_TrqLimitation','DMC_GenErr','DMC_SensorWarning','DMC_SlewrateLim','DMC_TempMotorLim','DMC_Running','DMC_Ready'},'SgnStartBit',{0,16,32,48,49,50,51,52,53,54,55,56,57,58,60,61,62,63},'SgnLength',{16,16,16,1,1,1,1,1,1,1,1,1,1,1,1,1,1,1},'SgnType',{'standard','standard','standard','standard','standard','standard','standard','standard','standard','standard','standard','standard','standard','standard','standard','standard','standard','standard'},'ModeValue',{-1,-1,-1,-1,-1,-1,-1,-1,-1,-1,-1,-1,-1,-1,-1,-1,-1,-1},'DataType',{['signed int'],['signed int'],['signed int'],['unsigned int'],['unsigned int'],['unsigned int'],['unsigned int'],['unsigned int'],['unsigned int'],['unsigned int'],['unsigned int'],['unsigned int'],['unsigned int'],['unsigned int'],['unsigned int'],['unsigned int'],['unsigned int'],['unsigned int']},'ByteLayout',{['motorola back.'],['motorola back.'],['motorola back.'],['motorola back.'],['motorola back.'],['motorola back.'],['motorola back.'],['motorola back.'],['motorola back.'],['motorola back.'],['motorola back.'],['motorola back.'],['motorola back.'],['motorola back.'],['motorola back.'],['motorola back.'],['motorola back.'],['motorola back.']},'Factor',{1,0.01,0.01,1,1,1,1,1,1,1,1,1,1,1,1,1,1,1},'Offset',{0,0,0,0,0,0,0,0,0,0,0,0,0,0,0,0,0,0},'SLDataType',{'SS_DOUBLE','SS_DOUBLE','SS_DOUBLE','SS_DOUBLE','SS_DOUBLE','SS_DOUBLE','SS_DOUBLE','SS_DOUBLE','SS_DOUBLE','SS_DOUBLE','SS_DOUBLE','SS_DOUBLE','SS_DOUBLE','SS_DOUBLE','SS_DOUBLE','SS_DOUBLE','SS_DOUBLE','SS_DOUBLE'}),'StatusSelected','yes','TimeSelected','no','DeltaTimeSelected','no','BytePortSelected','no','MessageLengthSelected','no','TriggerPort',struct('Selected','no','TriggerType',0),'UserCoding',struct('Selected','no','InterfaceFile','UserDecodingFile','FcnName','UserDecodeFcn','InportSelected','no','InportWidth',1,'OutportSelected','no','OutportWidth',1),'EnablePortSelected','no','UseRXService','no','BoardType','DS1','BoardNo',2,'ControllerNo',1),'OFF',[]}},'TLCFileName',{{'rtican_rx_message','OFF',[]}})  RTISFcnParameters=struct('SFcnRTICANMessage','struct','TLCFileName','char')  RTIBlockParaDefault=struct('BoardTypeNo',4302,'BoardNo',1,'ChannelNo',1,'Parameters',struct('DataFileSupport',struct('DataFileSelectedMaster',0,'DataFileSelectedLocal',0,'DataFileName','','DataFileDate','','SelectedFile',['<no file selected>']),'Options',struct('StatusSelected',1,'TimeSelected',1,'DeltaTimeSelected',1,'BytePortSelected',0,'MessageLengthSelected',0,'TriggerPort',struct('Selected',0,'TriggerType','rising'),'UserCoding',struct('Selected',0,'InterfaceFile','UserDecodingFile','FcnName','UserDecodeFcn','InportSelected',0,'InportWidth',1,'OutportSelected',0,'OutportWidth',1),'EnablePortSelected',0,'SignalOnPortnameSelected',1,'UseRXService',0),'Message',struct('MsgOnBlocknameSelected',0,'MsgName',['RX Message'],'MsgIdFormat',0,'MsgId',100,'MsgLength',8,'NumSignals',1,'SampleTime',-1,'Signal',struct('SgnName',['RX signal'],'SgnStartBit',0,'SgnLength',8,'SgnType',0,'ModeValue',-1,'DataType',0,'SLDataType','SS_DOUBLE','ByteLayout',0,'Factor',1,'Offset',0,'Min',0,'Max',255,'SgnComment',{{}},'SgnUnit',''),'MsgIdNumFormat',0,'MsgComment',{{''}}),'Version',1.2,'general',struct('isFromLib',1)),'GroupId',struct('Group',{{'RTICAN'}},'No',1,'Behavior',{{'NAMECHANGE'}},'BlockType',{{'SINK'}},'NameChangeFlag',0),'SFcnRTICANMessage',struct('MsgType','RX','MsgName',['RX Message'],'MsgIdFormat','STD','MsgId',100,'MsgLength',8,'NumSignals',1,'SampleTime',-1,'Signal',struct('SgnName',['RX signal'],'SgnStartBit',0,'SgnLength',8,'SgnType','standard','ModeValue',-1,'DataType',['unsigned int'],'ByteLayout',['little endian'],'SLDataType','SS_DOUBLE','Factor',1,'Offset',0),'StatusSelected','yes','TimeSelected','yes','DeltaTimeSelected','yes','BytePortSelected','no','MessageLengthSelected','no','EnablePortSelected','no','UserCoding',struct('Selected','no','InterfaceFile','UserDecodingFile','FcnName','UserDecodeFcn','InportSelected','no','InportWidth',1,'OutportSelected','no','OutportWidth',1),'TriggerPort',struct('Selected','no','TriggerType','rising'),'UseRXService','no','BoardType','DS4302','BoardNo',1,'ControllerNo',1,'SFcnPortType','Scalar'),'TLCFileName','rtican_rx_message')
      settings: AttributesFormatString=Group Id: RTICAN3\n
  DMC2_TRQS2 : rtican/RTICAN Receive (RX)   Reserved1=[]  Reserved2=[]  Reserved3=[]  Reserved4=[]  SfcnMessage=[]  Msg_Struct=[]  BoardTypeNo=[]  BoardNo=[]  ChannelNo=[]  Parameters=[]  DialogFcn=[]  UnitName=[]  Revision=[]  UnitValues=[]  DSProperties=struct('RTI',struct('Version',uint32(5),'BlockType',struct('isSLSource',uint8(1),'isSLSink',uint8(1),'isHWSource',uint8(0),'isHWSink',uint8(0),'isSetup',uint8(0),'isInline',uint8(1),'isNonInline',uint8(0),'isInterrupt',uint8(0),'isChannelwise',uint8(0)),'IOBoardType','RTICAN','UnitType','MESSAGE','Identifier','RX','DialogType','MSVC','BlockSet','RTICAN','SlaveProcessor','CAN'))  RTIBlockInterface=struct('OutputPortsWidth',int32([1 1 1]),'OutputPortsActive',[1 1 1],'OutputPortsName',{{'DMC_ActiveLimit','DMC_TrqMin','DMC_TrqMax'}},'OutputPortsDataType',{{'SS_DOUBLE','SS_DOUBLE','SS_DOUBLE'}},'OutputPortsLabel',{{'DMC_ActiveLimit','DMC_TrqMin','DMC_TrqMax'}},'OutputPortsLabelMode','ON','InputPortsWidth',int32(0),'InputPortsActive',0,'DialogFcn','rtican_message_interface_gui','BlockDisplay',{{'','center'}},'IconTransparency','on','ParameterTunableNames',{{}},'InitLevel',3,'BlockName',struct('Token',{{'DMC_TRQS2'}}),'SampleTime',{{-1}},'TriggerPort',{{'none'}},'EnablePort',{{'none'}})  RTIBlockParameters=struct('BoardTypeNo',{{1,'OFF',[]}},'BoardNo',{{1,'ON',[1 16]}},'ChannelNo',{{1,'ON',[1 2]}},'Parameters',{{struct('DataFileSupport',struct('DataFileSelectedMaster',1,'DataFileSelectedLocal',0,'DataFileName','c:\users\powertrain_software\desktop\brusa_02-01-02_rev02-2\documentation\dmc5_can_spec_3.9.dbc|','DataFileDate',{{{['14-dec-2011 16:00:26']}}},'SelectedFile',['<no file selected>']),'Options',struct('StatusSelected',0,'TimeSelected',0,'DeltaTimeSelected',0,'BytePortSelected',0,'MessageLengthSelected',0,'TriggerPort',struct('Selected',0,'TriggerType',0),'UserCoding',struct('Selected',0,'InterfaceFile','UserDecodingFile','FcnName','UserDecodeFcn','InportSelected',0,'InportWidth',1,'OutportSelected',0,'OutportWidth',1),'EnablePortSelected',0,'SignalOnPortnameSelected',1,'UseRXService',0),'Message',struct('MsgOnBlocknameSelected',1,'MsgName','DMC2_TRQS2','MsgIdFormat',0,'MsgId',619,'MsgLength',8,'NumSignals',3,'SampleTime',-1,'Signal',struct('SgnName',{'DMC_ActiveLimit','DMC_TrqMin','DMC_TrqMax'},'SgnStartBit',{24,32,48},'SgnLength',{8,16,16},'SgnType',{0,0,0},'ModeValue',{-1,-1,-1},'DataType',{0,1,1},'ByteLayout',{2,2,2},'Factor',{1,0.01,0.01},'Offset',{0,0,0},'SgnComment',{{['state number of active limiter']},{['min negative available torque']},{['max positive available torque']}},'SgnUnit',{'','Nm','Nm'},'Min',{0,-327.68,-327.68},'Max',{255,327.67,327.67},'SLDataType',{'SS_DOUBLE','SS_DOUBLE','SS_DOUBLE'}),'MsgIdNumFormat',1,'MsgComment',{{''}}),'Version',1.2,'general',struct('isFromLib',0)),'OFF',[]}},'GroupId',{{struct('Group',{{'RTICAN'}},'No',1,'Behavior',{{'NAMECHANGE'}},'BlockType',{{'SINK'}},'NameChangeFlag',0),'OFF',[]}},'SFcnRTICANMessage',{{struct('MsgType','RX','SFcnPortType','Scalar','MsgName','DMC2_TRQS2','MsgIdFormat','STD','MsgId',619,'MsgLength',8,'NumSignals',3,'SampleTime',-1,'Signal',struct('SgnName',{'DMC_ActiveLimit','DMC_TrqMin','DMC_TrqMax'},'SgnStartBit',{24,32,48},'SgnLength',{8,16,16},'SgnType',{'standard','standard','standard'},'ModeValue',{-1,-1,-1},'DataType',{['unsigned int'],['signed int'],['signed int']},'ByteLayout',{['motorola back.'],['motorola back.'],['motorola back.']},'Factor',{1,0.01,0.01},'Offset',{0,0,0},'SLDataType',{'SS_DOUBLE','SS_DOUBLE','SS_DOUBLE'}),'StatusSelected','no','TimeSelected','no','DeltaTimeSelected','no','BytePortSelected','no','MessageLengthSelected','no','TriggerPort',struct('Selected','no','TriggerType',0),'UserCoding',struct('Selected','no','InterfaceFile','UserDecodingFile','FcnName','UserDecodeFcn','InportSelected','no','InportWidth',1,'OutportSelected','no','OutportWidth',1),'EnablePortSelected','no','UseRXService','no','BoardType','DS1','BoardNo',2,'ControllerNo',2),'OFF',[]}},'TLCFileName',{{'rtican_rx_message','OFF',[]}})  RTISFcnParameters=struct('SFcnRTICANMessage','struct','TLCFileName','char')  RTIBlockParaDefault=struct('BoardTypeNo',4302,'BoardNo',1,'ChannelNo',1,'Parameters',struct('DataFileSupport',struct('DataFileSelectedMaster',0,'DataFileSelectedLocal',0,'DataFileName','','DataFileDate','','SelectedFile',['<no file selected>']),'Options',struct('StatusSelected',1,'TimeSelected',1,'DeltaTimeSelected',1,'BytePortSelected',0,'MessageLengthSelected',0,'TriggerPort',struct('Selected',0,'TriggerType','rising'),'UserCoding',struct('Selected',0,'InterfaceFile','UserDecodingFile','FcnName','UserDecodeFcn','InportSelected',0,'InportWidth',1,'OutportSelected',0,'OutportWidth',1),'EnablePortSelected',0,'SignalOnPortnameSelected',1,'UseRXService',0),'Message',struct('MsgOnBlocknameSelected',0,'MsgName',['RX Message'],'MsgIdFormat',0,'MsgId',100,'MsgLength',8,'NumSignals',1,'SampleTime',-1,'Signal',struct('SgnName',['RX signal'],'SgnStartBit',0,'SgnLength',8,'SgnType',0,'ModeValue',-1,'DataType',0,'SLDataType','SS_DOUBLE','ByteLayout',0,'Factor',1,'Offset',0,'Min',0,'Max',255,'SgnComment',{{}},'SgnUnit',''),'MsgIdNumFormat',0,'MsgComment',{{''}}),'Version',1.2,'general',struct('isFromLib',1)),'GroupId',struct('Group',{{'RTICAN'}},'No',1,'Behavior',{{'NAMECHANGE'}},'BlockType',{{'SINK'}},'NameChangeFlag',0),'SFcnRTICANMessage',struct('MsgType','RX','MsgName',['RX Message'],'MsgIdFormat','STD','MsgId',100,'MsgLength',8,'NumSignals',1,'SampleTime',-1,'Signal',struct('SgnName',['RX signal'],'SgnStartBit',0,'SgnLength',8,'SgnType','standard','ModeValue',-1,'DataType',['unsigned int'],'ByteLayout',['little endian'],'SLDataType','SS_DOUBLE','Factor',1,'Offset',0),'StatusSelected','yes','TimeSelected','yes','DeltaTimeSelected','yes','BytePortSelected','no','MessageLengthSelected','no','EnablePortSelected','no','UserCoding',struct('Selected','no','InterfaceFile','UserDecodingFile','FcnName','UserDecodeFcn','InportSelected','no','InportWidth',1,'OutportSelected','no','OutportWidth',1),'TriggerPort',struct('Selected','no','TriggerType','rising'),'UseRXService','no','BoardType','DS4302','BoardNo',1,'ControllerNo',1,'SFcnPortType','Scalar'),'TLCFileName','rtican_rx_message')
      settings: AttributesFormatString=Group Id: RTICAN1\n
  DMC_ACTV : rtican/RTICAN Receive (RX)   Reserved1=[]  Reserved2=[]  Reserved3=[]  Reserved4=[]  SfcnMessage=[]  Msg_Struct=[]  BoardTypeNo=[]  BoardNo=[]  ChannelNo=[]  Parameters=[]  DialogFcn=[]  UnitName=[]  Revision=[]  UnitValues=[]  DSProperties=struct('RTI',struct('Version',uint32(5),'BlockType',struct('isSLSource',uint8(1),'isSLSink',uint8(1),'isHWSource',uint8(0),'isHWSink',uint8(0),'isSetup',uint8(0),'isInline',uint8(1),'isNonInline',uint8(0),'isInterrupt',uint8(0),'isChannelwise',uint8(0)),'IOBoardType','RTICAN','UnitType','MESSAGE','Identifier','RX','DialogType','MSVC','BlockSet','RTICAN','SlaveProcessor','CAN'))  RTIBlockInterface=struct('OutputPortsWidth',int32([1 1 1 1]),'OutputPortsActive',[1 1 1 1],'OutputPortsName',{{'DMC_MechPwr','DMC_AcCurrAct','DMC_DcCurrAct','DMC_DcVltAct'}},'OutputPortsDataType',{{'SS_DOUBLE','SS_DOUBLE','SS_DOUBLE','SS_DOUBLE'}},'OutputPortsLabel',{{'DMC_MechPwr','DMC_AcCurrAct','DMC_DcCurrAct','DMC_DcVltAct'}},'OutputPortsLabelMode','ON','InputPortsWidth',int32(0),'InputPortsActive',0,'DialogFcn','rtican_message_interface_gui','BlockDisplay',{{'','center'}},'IconTransparency','on','ParameterTunableNames',{{}},'InitLevel',3,'BlockName',struct('Token',{{'DMC_ACTV'}}),'SampleTime',{{-1}},'TriggerPort',{{'none'}},'EnablePort',{{'none'}})  RTIBlockParameters=struct('BoardTypeNo',{{1,'OFF',[]}},'BoardNo',{{1,'ON',[1 16]}},'ChannelNo',{{2,'ON',[1 2]}},'Parameters',{{struct('DataFileSupport',struct('DataFileSelectedMaster',1,'DataFileSelectedLocal',1,'DataFileName','c:\users\powertrain_software\desktop\brusa_02-01-02_rev02-2\documentation\dmc5_can_spec_3.9.dbc|','DataFileDate',{{{['14-dec-2011 16:00:26']}}},'SelectedFile','..\brusa_02-01-02_rev02-2\documentation\dmc5_can_spec_3.9.dbc'),'Options',struct('StatusSelected',0,'TimeSelected',0,'DeltaTimeSelected',0,'BytePortSelected',0,'MessageLengthSelected',0,'TriggerPort',struct('Selected',0,'TriggerType',0),'UserCoding',struct('Selected',0,'InterfaceFile','UserDecodingFile','FcnName','UserDecodeFcn','InportSelected',0,'InportWidth',1,'OutportSelected',0,'OutportWidth',1),'EnablePortSelected',0,'SignalOnPortnameSelected',1,'UseRXService',0),'Message',struct('MsgOnBlocknameSelected',1,'MsgName','DMC_ACTV','MsgIdFormat',0,'MsgId',601,'MsgLength',8,'NumSignals',4,'SampleTime',-1,'Signal',struct('SgnName',{'DMC_MechPwr','DMC_AcCurrAct','DMC_DcCurrAct','DMC_DcVltAct'},'SgnStartBit',{0,16,32,48},'SgnLength',{16,16,16,16},'SgnType',{0,0,0,0},'ModeValue',{-1,-1,-1,-1},'DataType',{1,0,1,0},'ByteLayout',{2,2,2,2},'Factor',{16,0.25,0.1,0.1},'Offset',{0,0,0,0},'SgnComment',{{['DMC_MechPwr has new scaling compared to older DMC5 SW Versions!']},{['actual AC current peak value']},{['actual dc current']},{['actual dc voltage']}},'SgnUnit',{'W','A','A','V'},'Min',{-524288,0,-3276.8,0},'Max',{524272,16383.75,3276.7,6553.5},'SLDataType',{'SS_DOUBLE','SS_DOUBLE','SS_DOUBLE','SS_DOUBLE'}),'MsgIdNumFormat',1,'MsgComment',{{''}}),'Version',1.2,'general',struct('isFromLib',0)),'OFF',[]}},'GroupId',{{struct('Group',{{'RTICAN'}},'No',2,'Behavior',{{'NAMECHANGE'}},'BlockType',{{'SINK'}},'NameChangeFlag',0),'OFF',[]}},'SFcnRTICANMessage',{{struct('MsgType','RX','SFcnPortType','Scalar','MsgName','DMC_ACTV','MsgIdFormat','STD','MsgId',601,'MsgLength',8,'NumSignals',4,'SampleTime',-1,'Signal',struct('SgnName',{'DMC_MechPwr','DMC_AcCurrAct','DMC_DcCurrAct','DMC_DcVltAct'},'SgnStartBit',{0,16,32,48},'SgnLength',{16,16,16,16},'SgnType',{'standard','standard','standard','standard'},'ModeValue',{-1,-1,-1,-1},'DataType',{['signed int'],['unsigned int'],['signed int'],['unsigned int']},'ByteLayout',{['motorola back.'],['motorola back.'],['motorola back.'],['motorola back.']},'Factor',{16,0.25,0.1,0.1},'Offset',{0,0,0,0},'SLDataType',{'SS_DOUBLE','SS_DOUBLE','SS_DOUBLE','SS_DOUBLE'}),'StatusSelected','no','TimeSelected','no','DeltaTimeSelected','no','BytePortSelected','no','MessageLengthSelected','no','TriggerPort',struct('Selected','no','TriggerType',0),'UserCoding',struct('Selected','no','InterfaceFile','UserDecodingFile','FcnName','UserDecodeFcn','InportSelected','no','InportWidth',1,'OutportSelected','no','OutportWidth',1),'EnablePortSelected','no','UseRXService','no','BoardType','DS1','BoardNo',1,'ControllerNo',2),'OFF',[]}},'TLCFileName',{{'rtican_rx_message','OFF',[]}})  RTISFcnParameters=struct('SFcnRTICANMessage','struct','TLCFileName','char')  RTIBlockParaDefault=struct('BoardTypeNo',4302,'BoardNo',1,'ChannelNo',1,'Parameters',struct('DataFileSupport',struct('DataFileSelectedMaster',0,'DataFileSelectedLocal',0,'DataFileName','','DataFileDate','','SelectedFile',['<no file selected>']),'Options',struct('StatusSelected',1,'TimeSelected',1,'DeltaTimeSelected',1,'BytePortSelected',0,'MessageLengthSelected',0,'TriggerPort',struct('Selected',0,'TriggerType','rising'),'UserCoding',struct('Selected',0,'InterfaceFile','UserDecodingFile','FcnName','UserDecodeFcn','InportSelected',0,'InportWidth',1,'OutportSelected',0,'OutportWidth',1),'EnablePortSelected',0,'SignalOnPortnameSelected',1,'UseRXService',0),'Message',struct('MsgOnBlocknameSelected',0,'MsgName',['RX Message'],'MsgIdFormat',0,'MsgId',100,'MsgLength',8,'NumSignals',1,'SampleTime',-1,'Signal',struct('SgnName',['RX signal'],'SgnStartBit',0,'SgnLength',8,'SgnType',0,'ModeValue',-1,'DataType',0,'SLDataType','SS_DOUBLE','ByteLayout',0,'Factor',1,'Offset',0,'Min',0,'Max',255,'SgnComment',{{}},'SgnUnit',''),'MsgIdNumFormat',0,'MsgComment',{{''}}),'Version',1.2,'general',struct('isFromLib',1)),'GroupId',struct('Group',{{'RTICAN'}},'No',1,'Behavior',{{'NAMECHANGE'}},'BlockType',{{'SINK'}},'NameChangeFlag',0),'SFcnRTICANMessage',struct('MsgType','RX','MsgName',['RX Message'],'MsgIdFormat','STD','MsgId',100,'MsgLength',8,'NumSignals',1,'SampleTime',-1,'Signal',struct('SgnName',['RX signal'],'SgnStartBit',0,'SgnLength',8,'SgnType','standard','ModeValue',-1,'DataType',['unsigned int'],'ByteLayout',['little endian'],'SLDataType','SS_DOUBLE','Factor',1,'Offset',0),'StatusSelected','yes','TimeSelected','yes','DeltaTimeSelected','yes','BytePortSelected','no','MessageLengthSelected','no','EnablePortSelected','no','UserCoding',struct('Selected','no','InterfaceFile','UserDecodingFile','FcnName','UserDecodeFcn','InportSelected','no','InportWidth',1,'OutportSelected','no','OutportWidth',1),'TriggerPort',struct('Selected','no','TriggerType','rising'),'UseRXService','no','BoardType','DS4302','BoardNo',1,'ControllerNo',1,'SFcnPortType','Scalar'),'TLCFileName','rtican_rx_message')
      settings: AttributesFormatString=Group Id: RTICAN2\n
  DMC_ERR : rtican/RTICAN Receive (RX)   Reserved1=[]  Reserved2=[]  Reserved3=[]  Reserved4=[]  SfcnMessage=[]  Msg_Struct=[]  BoardTypeNo=[]  BoardNo=[]  ChannelNo=[]  Parameters=[]  DialogFcn=[]  UnitName=[]  Revision=[]  UnitValues=[]  DSProperties=struct('RTI',struct('Version',uint32(5),'BlockType',struct('isSLSource',uint8(1),'isSLSink',uint8(1),'isHWSource',uint8(0),'isHWSink',uint8(0),'isSetup',uint8(0),'isInline',uint8(1),'isNonInline',uint8(0),'isInterrupt',uint8(0),'isChannelwise',uint8(0)),'IOBoardType','RTICAN','UnitType','MESSAGE','Identifier','RX','DialogType','MSVC','BlockSet','RTICAN','SlaveProcessor','CAN'))  RTIBlockInterface=struct('OutputPortsWidth',int32([1 1 1 1 1 1 1 1 1 1 1 1 1 1 1 1 1 1 1 1 1 1 1 1 1 1 1 1 1 1 1 1 1 1 1 1 1 1]),'OutputPortsActive',[1 1 1 1 1 1 1 1 1 1 1 1 1 1 1 1 1 1 1 1 1 1 1 1 1 1 1 1 1 1 1 1 1 1 1 1 1 1],'OutputPortsName',{{'DMC_I_SystemCheck','DMC_I_ExtAw2','DMC_I_ExtAw1','DMC_I_OscLim_Active','DMC_W_DriverSD','DMC_W_PowerMismatch','DMC_W_SpeedSensor','DMC_W_HvUndervoltage','DMC_W_ModMaxLim','DMC_W_TempSensor','DMC_E_AN_IN','DMC_E_DriverSD','DMC_E_PowerMismatch','DMC_E_CanCtrl2MsgLost','DMC_E_MotEEPROM','DMC_E_Storage','DMC_E_KL15Lost','DMC_E_CanComStartup','DMC_E_IntSupply','DMC_E_AC_Overcurr','DMC_E_OS_Trap','DMC_CompatibilityWarnings','DMC_E_SpdSensSupply','DMC_E_SpeedSensor','DMC_E_CanLimMsgInvalid','DMC_E_CanCtrlMsgInvalid','DMC_E_CanLimMsgLost','DMC_E_SkyVlt','DMC_E_VltMeas','DMC_E_ShortCircuit','DMC_E_CanCtrlMsgLost','DMC_E_TempDmc','DMC_E_TempMot','DMC_E_Speed','DMC_E_UV','DMC_E_OV','DMC_E_DcCurr','DMC_E_Init'}},'OutputPortsDataType',{{'SS_DOUBLE','SS_DOUBLE','SS_DOUBLE','SS_DOUBLE','SS_DOUBLE','SS_DOUBLE','SS_DOUBLE','SS_DOUBLE','SS_DOUBLE','SS_DOUBLE','SS_DOUBLE','SS_DOUBLE','SS_DOUBLE','SS_DOUBLE','SS_DOUBLE','SS_DOUBLE','SS_DOUBLE','SS_DOUBLE','SS_DOUBLE','SS_DOUBLE','SS_DOUBLE','SS_DOUBLE','SS_DOUBLE','SS_DOUBLE','SS_DOUBLE','SS_DOUBLE','SS_DOUBLE','SS_DOUBLE','SS_DOUBLE','SS_DOUBLE','SS_DOUBLE','SS_DOUBLE','SS_DOUBLE','SS_DOUBLE','SS_DOUBLE','SS_DOUBLE','SS_DOUBLE','SS_DOUBLE'}},'OutputPortsLabel',{{'DMC_I_SystemCheck','DMC_I_ExtAw2','DMC_I_ExtAw1','DMC_I_OscLim_Active','DMC_W_DriverSD','DMC_W_PowerMismatch','DMC_W_SpeedSensor','DMC_W_HvUndervoltage','DMC_W_ModMaxLim','DMC_W_TempSensor','DMC_E_AN_IN','DMC_E_DriverSD','DMC_E_PowerMismatch','DMC_E_CanCtrl2MsgLost','DMC_E_MotEEPROM','DMC_E_Storage','DMC_E_KL15Lost','DMC_E_CanComStartup','DMC_E_IntSupply','DMC_E_AC_Overcurr','DMC_E_OS_Trap','DMC_CompatibilityWarnings','DMC_E_SpdSensSupply','DMC_E_SpeedSensor','DMC_E_CanLimMsgInvalid','DMC_E_CanCtrlMsgInvalid','DMC_E_CanLimMsgLost','DMC_E_SkyVlt','DMC_E_VltMeas','DMC_E_ShortCircuit','DMC_E_CanCtrlMsgLost','DMC_E_TempDmc','DMC_E_TempMot','DMC_E_Speed','DMC_E_UV','DMC_E_OV','DMC_E_DcCurr','DMC_E_Init'}},'OutputPortsLabelMode','ON','InputPortsWidth',int32(0),'InputPortsActive',0,'DialogFcn','rtican_message_interface_gui','BlockDisplay',{{'','center'}},'IconTransparency','on','ParameterTunableNames',{{}},'InitLevel',3,'BlockName',struct('Token',{{'DMC_ERR'}}),'SampleTime',{{-1}},'TriggerPort',{{'none'}},'EnablePort',{{'none'}})  RTIBlockParameters=struct('BoardTypeNo',{{1,'OFF',[]}},'BoardNo',{{1,'ON',[1 16]}},'ChannelNo',{{2,'ON',[1 2]}},'Parameters',{{struct('DataFileSupport',struct('DataFileSelectedMaster',1,'DataFileSelectedLocal',1,'DataFileName','c:\users\powertrain_software\desktop\brusa_02-01-02_rev02-2\documentation\dmc5_can_spec_3.9.dbc|','DataFileDate',{{{['14-dec-2011 16:00:26']}}},'SelectedFile','..\brusa_02-01-02_rev02-2\documentation\dmc5_can_spec_3.9.dbc'),'Options',struct('StatusSelected',0,'TimeSelected',0,'DeltaTimeSelected',0,'BytePortSelected',0,'MessageLengthSelected',0,'TriggerPort',struct('Selected',0,'TriggerType',0),'UserCoding',struct('Selected',0,'InterfaceFile','UserDecodingFile','FcnName','UserDecodeFcn','InportSelected',0,'InportWidth',1,'OutportSelected',0,'OutportWidth',1),'EnablePortSelected',0,'SignalOnPortnameSelected',1,'UseRXService',0),'Message',struct('MsgOnBlocknameSelected',1,'MsgName','DMC_ERR','MsgIdFormat',0,'MsgId',602,'MsgLength',8,'NumSignals',38,'SampleTime',-1,'Signal',struct('SgnName',{'DMC_I_SystemCheck','DMC_I_ExtAw2','DMC_I_ExtAw1','DMC_I_OscLim_Active','DMC_W_DriverSD','DMC_W_PowerMismatch','DMC_W_SpeedSensor','DMC_W_HvUndervoltage','DMC_W_ModMaxLim','DMC_W_TempSensor','DMC_E_AN_IN','DMC_E_DriverSD','DMC_E_PowerMismatch','DMC_E_CanCtrl2MsgLost','DMC_E_MotEEPROM','DMC_E_Storage','DMC_E_KL15Lost','DMC_E_CanComStartup','DMC_E_IntSupply','DMC_E_AC_Overcurr','DMC_E_OS_Trap','DMC_CompatibilityWarnings','DMC_E_SpdSensSupply','DMC_E_SpeedSensor','DMC_E_CanLimMsgInvalid','DMC_E_CanCtrlMsgInvalid','DMC_E_CanLimMsgLost','DMC_E_SkyVlt','DMC_E_VltMeas','DMC_E_ShortCircuit','DMC_E_CanCtrlMsgLost','DMC_E_TempDmc','DMC_E_TempMot','DMC_E_Speed','DMC_E_UV','DMC_E_OV','DMC_E_DcCurr','DMC_E_Init'},'SgnStartBit',{0,1,2,3,10,11,12,13,14,15,16,22,23,24,25,26,27,28,29,30,31,32,48,49,50,51,52,53,54,55,56,57,58,59,60,61,62,63},'SgnLength',{1,1,1,1,1,1,1,1,1,1,1,1,1,1,1,1,1,1,1,1,1,16,1,1,1,1,1,1,1,1,1,1,1,1,1,1,1,1},'SgnType',{0,0,0,0,0,0,0,0,0,0,0,0,0,0,0,0,0,0,0,0,0,0,0,0,0,0,0,0,0,0,0,0,0,0,0,0,0,0},'ModeValue',{-1,-1,-1,-1,-1,-1,-1,-1,-1,-1,-1,-1,-1,-1,-1,-1,-1,-1,-1,-1,-1,-1,-1,-1,-1,-1,-1,-1,-1,-1,-1,-1,-1,-1,-1,-1,-1,-1},'DataType',{0,0,0,0,0,0,0,0,0,0,0,0,0,0,0,0,0,0,0,0,0,0,0,0,0,0,0,0,0,0,0,0,0,0,0,0,0,0},'ByteLayout',{2,2,2,2,2,2,2,2,2,2,2,2,2,2,2,2,2,2,2,2,2,2,2,2,2,2,2,2,2,2,2,2,2,2,2,2,2,2},'Factor',{1,1,1,1,1,1,1,1,1,1,1,1,1,1,1,1,1,1,1,1,1,1,1,1,1,1,1,1,1,1,1,1,1,1,1,1,1,1},'Offset',{0,0,0,0,0,0,0,0,0,0,0,0,0,0,0,0,0,0,0,0,0,0,0,0,0,0,0,0,0,0,0,0,0,0,0,0,0,0},'SgnComment',{{['warnings are described in seperate document']},{['warnings are described in seperate document']},{['warnings are described in seperate document']},{['warnings are described in seperate document']},{['errors are described in seperate document']},{['warnings are described in seperate document']},{['warnings are described in seperate document']},{['warnings are described in seperate document']},{['warnings are described in seperate document']},{['warnings are described in seperate document']},{['errors are described in seperate document']},{['errors are described in seperate document']},{['errors are described in seperate document']},{['errors are described in seperate document']},{['errors are described in seperate document']},{['errors are described in seperate document']},{['errors are described in seperate document']},{['errors are described in seperate document']},{['errors are described in seperate document']},{['errors are described in seperate document']},{['errors are described in seperate document']},{['Warning Bitmap CAN Matrix <= 3.6 is sent at this Position']},{['errors are described in seperate document']},{['errors are described in seperate document']},{['errors are described in seperate document']},{['errors are described in seperate document']},{['errors are described in seperate document']},{['errors are described in seperate document']},{['errors are described in seperate document']},{['errors are described in seperate document']},{['errors are described in seperate document']},{['errors are described in seperate document']},{['errors are described in seperate document']},{['errors are described in seperate document']},{['errors are described in seperate document']},{['errors are described in seperate document']},{['errors are described in seperate document']},{['errors are described in seperate document']}},'SgnUnit',{'','','','','','','','','','','','','','','','','','','','','','','','','','','','','','','','','','','','','',''},'Min',{0,0,0,0,0,0,0,0,0,0,0,0,0,0,0,0,0,0,0,0,0,0,0,0,0,0,0,0,0,0,0,0,0,0,0,0,0,0},'Max',{0,0,0,0,0,0,0,0,0,0,0,0,0,0,0,0,0,0,0,0,0,0,0,0,0,0,0,0,0,0,0,0,0,0,0,0,0,0},'SLDataType',{'SS_DOUBLE','SS_DOUBLE','SS_DOUBLE','SS_DOUBLE','SS_DOUBLE','SS_DOUBLE','SS_DOUBLE','SS_DOUBLE','SS_DOUBLE','SS_DOUBLE','SS_DOUBLE','SS_DOUBLE','SS_DOUBLE','SS_DOUBLE','SS_DOUBLE','SS_DOUBLE','SS_DOUBLE','SS_DOUBLE','SS_DOUBLE','SS_DOUBLE','SS_DOUBLE','SS_DOUBLE','SS_DOUBLE','SS_DOUBLE','SS_DOUBLE','SS_DOUBLE','SS_DOUBLE','SS_DOUBLE','SS_DOUBLE','SS_DOUBLE','SS_DOUBLE','SS_DOUBLE','SS_DOUBLE','SS_DOUBLE','SS_DOUBLE','SS_DOUBLE','SS_DOUBLE','SS_DOUBLE'}),'MsgIdNumFormat',0,'MsgComment',{{''}}),'Version',1.2,'general',struct('isFromLib',0)),'OFF',[]}},'GroupId',{{struct('Group',{{'RTICAN'}},'No',2,'Behavior',{{'NAMECHANGE'}},'BlockType',{{'SINK'}},'NameChangeFlag',0),'OFF',[]}},'SFcnRTICANMessage',{{struct('MsgType','RX','SFcnPortType','Scalar','MsgName','DMC_ERR','MsgIdFormat','STD','MsgId',602,'MsgLength',8,'NumSignals',38,'SampleTime',-1,'Signal',struct('SgnName',{'DMC_I_SystemCheck','DMC_I_ExtAw2','DMC_I_ExtAw1','DMC_I_OscLim_Active','DMC_W_DriverSD','DMC_W_PowerMismatch','DMC_W_SpeedSensor','DMC_W_HvUndervoltage','DMC_W_ModMaxLim','DMC_W_TempSensor','DMC_E_AN_IN','DMC_E_DriverSD','DMC_E_PowerMismatch','DMC_E_CanCtrl2MsgLost','DMC_E_MotEEPROM','DMC_E_Storage','DMC_E_KL15Lost','DMC_E_CanComStartup','DMC_E_IntSupply','DMC_E_AC_Overcurr','DMC_E_OS_Trap','DMC_CompatibilityWarnings','DMC_E_SpdSensSupply','DMC_E_SpeedSensor','DMC_E_CanLimMsgInvalid','DMC_E_CanCtrlMsgInvalid','DMC_E_CanLimMsgLost','DMC_E_SkyVlt','DMC_E_VltMeas','DMC_E_ShortCircuit','DMC_E_CanCtrlMsgLost','DMC_E_TempDmc','DMC_E_TempMot','DMC_E_Speed','DMC_E_UV','DMC_E_OV','DMC_E_DcCurr','DMC_E_Init'},'SgnStartBit',{0,1,2,3,10,11,12,13,14,15,16,22,23,24,25,26,27,28,29,30,31,32,48,49,50,51,52,53,54,55,56,57,58,59,60,61,62,63},'SgnLength',{1,1,1,1,1,1,1,1,1,1,1,1,1,1,1,1,1,1,1,1,1,16,1,1,1,1,1,1,1,1,1,1,1,1,1,1,1,1},'SgnType',{'standard','standard','standard','standard','standard','standard','standard','standard','standard','standard','standard','standard','standard','standard','standard','standard','standard','standard','standard','standard','standard','standard','standard','standard','standard','standard','standard','standard','standard','standard','standard','standard','standard','standard','standard','standard','standard','standard'},'ModeValue',{-1,-1,-1,-1,-1,-1,-1,-1,-1,-1,-1,-1,-1,-1,-1,-1,-1,-1,-1,-1,-1,-1,-1,-1,-1,-1,-1,-1,-1,-1,-1,-1,-1,-1,-1,-1,-1,-1},'DataType',{['unsigned int'],['unsigned int'],['unsigned int'],['unsigned int'],['unsigned int'],['unsigned int'],['unsigned int'],['unsigned int'],['unsigned int'],['unsigned int'],['unsigned int'],['unsigned int'],['unsigned int'],['unsigned int'],['unsigned int'],['unsigned int'],['unsigned int'],['unsigned int'],['unsigned int'],['unsigned int'],['unsigned int'],['unsigned int'],['unsigned int'],['unsigned int'],['unsigned int'],['unsigned int'],['unsigned int'],['unsigned int'],['unsigned int'],['unsigned int'],['unsigned int'],['unsigned int'],['unsigned int'],['unsigned int'],['unsigned int'],['unsigned int'],['unsigned int'],['unsigned int']},'ByteLayout',{['motorola back.'],['motorola back.'],['motorola back.'],['motorola back.'],['motorola back.'],['motorola back.'],['motorola back.'],['motorola back.'],['motorola back.'],['motorola back.'],['motorola back.'],['motorola back.'],['motorola back.'],['motorola back.'],['motorola back.'],['motorola back.'],['motorola back.'],['motorola back.'],['motorola back.'],['motorola back.'],['motorola back.'],['motorola back.'],['motorola back.'],['motorola back.'],['motorola back.'],['motorola back.'],['motorola back.'],['motorola back.'],['motorola back.'],['motorola back.'],['motorola back.'],['motorola back.'],['motorola back.'],['motorola back.'],['motorola back.'],['motorola back.'],['motorola back.'],['motorola back.']},'Factor',{1,1,1,1,1,1,1,1,1,1,1,1,1,1,1,1,1,1,1,1,1,1,1,1,1,1,1,1,1,1,1,1,1,1,1,1,1,1},'Offset',{0,0,0,0,0,0,0,0,0,0,0,0,0,0,0,0,0,0,0,0,0,0,0,0,0,0,0,0,0,0,0,0,0,0,0,0,0,0},'SLDataType',{'SS_DOUBLE','SS_DOUBLE','SS_DOUBLE','SS_DOUBLE','SS_DOUBLE','SS_DOUBLE','SS_DOUBLE','SS_DOUBLE','SS_DOUBLE','SS_DOUBLE','SS_DOUBLE','SS_DOUBLE','SS_DOUBLE','SS_DOUBLE','SS_DOUBLE','SS_DOUBLE','SS_DOUBLE','SS_DOUBLE','SS_DOUBLE','SS_DOUBLE','SS_DOUBLE','SS_DOUBLE','SS_DOUBLE','SS_DOUBLE','SS_DOUBLE','SS_DOUBLE','SS_DOUBLE','SS_DOUBLE','SS_DOUBLE','SS_DOUBLE','SS_DOUBLE','SS_DOUBLE','SS_DOUBLE','SS_DOUBLE','SS_DOUBLE','SS_DOUBLE','SS_DOUBLE','SS_DOUBLE'}),'StatusSelected','no','TimeSelected','no','DeltaTimeSelected','no','BytePortSelected','no','MessageLengthSelected','no','TriggerPort',struct('Selected','no','TriggerType',0),'UserCoding',struct('Selected','no','InterfaceFile','UserDecodingFile','FcnName','UserDecodeFcn','InportSelected','no','InportWidth',1,'OutportSelected','no','OutportWidth',1),'EnablePortSelected','no','UseRXService','no','BoardType','DS1','BoardNo',1,'ControllerNo',2),'OFF',[]}},'TLCFileName',{{'rtican_rx_message','OFF',[]}})  RTISFcnParameters=struct('SFcnRTICANMessage','struct','TLCFileName','char')  RTIBlockParaDefault=struct('BoardTypeNo',4302,'BoardNo',1,'ChannelNo',1,'Parameters',struct('DataFileSupport',struct('DataFileSelectedMaster',0,'DataFileSelectedLocal',0,'DataFileName','','DataFileDate','','SelectedFile',['<no file selected>']),'Options',struct('StatusSelected',1,'TimeSelected',1,'DeltaTimeSelected',1,'BytePortSelected',0,'MessageLengthSelected',0,'TriggerPort',struct('Selected',0,'TriggerType','rising'),'UserCoding',struct('Selected',0,'InterfaceFile','UserDecodingFile','FcnName','UserDecodeFcn','InportSelected',0,'InportWidth',1,'OutportSelected',0,'OutportWidth',1),'EnablePortSelected',0,'SignalOnPortnameSelected',1,'UseRXService',0),'Message',struct('MsgOnBlocknameSelected',0,'MsgName',['RX Message'],'MsgIdFormat',0,'MsgId',100,'MsgLength',8,'NumSignals',1,'SampleTime',-1,'Signal',struct('SgnName',['RX signal'],'SgnStartBit',0,'SgnLength',8,'SgnType',0,'ModeValue',-1,'DataType',0,'SLDataType','SS_DOUBLE','ByteLayout',0,'Factor',1,'Offset',0,'Min',0,'Max',255,'SgnComment',{{}},'SgnUnit',''),'MsgIdNumFormat',0,'MsgComment',{{''}}),'Version',1.2,'general',struct('isFromLib',1)),'GroupId',struct('Group',{{'RTICAN'}},'No',1,'Behavior',{{'NAMECHANGE'}},'BlockType',{{'SINK'}},'NameChangeFlag',0),'SFcnRTICANMessage',struct('MsgType','RX','MsgName',['RX Message'],'MsgIdFormat','STD','MsgId',100,'MsgLength',8,'NumSignals',1,'SampleTime',-1,'Signal',struct('SgnName',['RX signal'],'SgnStartBit',0,'SgnLength',8,'SgnType','standard','ModeValue',-1,'DataType',['unsigned int'],'ByteLayout',['little endian'],'SLDataType','SS_DOUBLE','Factor',1,'Offset',0),'StatusSelected','yes','TimeSelected','yes','DeltaTimeSelected','yes','BytePortSelected','no','MessageLengthSelected','no','EnablePortSelected','no','UserCoding',struct('Selected','no','InterfaceFile','UserDecodingFile','FcnName','UserDecodeFcn','InportSelected','no','InportWidth',1,'OutportSelected','no','OutportWidth',1),'TriggerPort',struct('Selected','no','TriggerType','rising'),'UseRXService','no','BoardType','DS4302','BoardNo',1,'ControllerNo',1,'SFcnPortType','Scalar'),'TLCFileName','rtican_rx_message')
      settings: AttributesFormatString=Group Id: RTICAN2\n
  DMC_TEMP : rtican/RTICAN Receive (RX)   Reserved1=[]  Reserved2=[]  Reserved3=[]  Reserved4=[]  SfcnMessage=[]  Msg_Struct=[]  BoardTypeNo=[]  BoardNo=[]  ChannelNo=[]  Parameters=[]  DialogFcn=[]  UnitName=[]  Revision=[]  UnitValues=[]  DSProperties=struct('RTI',struct('Version',uint32(5),'BlockType',struct('isSLSource',uint8(1),'isSLSink',uint8(1),'isHWSource',uint8(0),'isHWSink',uint8(0),'isSetup',uint8(0),'isInline',uint8(1),'isNonInline',uint8(0),'isInterrupt',uint8(0),'isChannelwise',uint8(0)),'IOBoardType','RTICAN','UnitType','MESSAGE','Identifier','RX','DialogType','MSVC','BlockSet','RTICAN','SlaveProcessor','CAN'))  RTIBlockInterface=struct('OutputPortsWidth',int32([1 1 1]),'OutputPortsActive',[1 1 1],'OutputPortsName',{{'DMC_TempSys','DMC_TempMot','DMC_TempInv'}},'OutputPortsDataType',{{'SS_DOUBLE','SS_DOUBLE','SS_DOUBLE'}},'OutputPortsLabel',{{'DMC_TempSys','DMC_TempMot','DMC_TempInv'}},'OutputPortsLabelMode','ON','InputPortsWidth',int32(0),'InputPortsActive',0,'DialogFcn','rtican_message_interface_gui','BlockDisplay',{{'','center'}},'IconTransparency','on','ParameterTunableNames',{{}},'InitLevel',3,'BlockName',struct('Token',{{'DMC_TEMP'}}),'SampleTime',{{-1}},'TriggerPort',{{'none'}},'EnablePort',{{'none'}})  RTIBlockParameters=struct('BoardTypeNo',{{1,'OFF',[]}},'BoardNo',{{1,'ON',[1 16]}},'ChannelNo',{{2,'ON',[1 2]}},'Parameters',{{struct('DataFileSupport',struct('DataFileSelectedMaster',1,'DataFileSelectedLocal',1,'DataFileName','c:\users\powertrain_software\desktop\brusa_02-01-02_rev02-2\documentation\dmc5_can_spec_3.9.dbc|','DataFileDate',{{{['14-dec-2011 16:00:26']}}},'SelectedFile','..\brusa_02-01-02_rev02-2\documentation\dmc5_can_spec_3.9.dbc'),'Options',struct('StatusSelected',0,'TimeSelected',0,'DeltaTimeSelected',0,'BytePortSelected',0,'MessageLengthSelected',0,'TriggerPort',struct('Selected',0,'TriggerType',0),'UserCoding',struct('Selected',0,'InterfaceFile','UserDecodingFile','FcnName','UserDecodeFcn','InportSelected',0,'InportWidth',1,'OutportSelected',0,'OutportWidth',1),'EnablePortSelected',0,'SignalOnPortnameSelected',1,'UseRXService',0),'Message',struct('MsgOnBlocknameSelected',1,'MsgName','DMC_TEMP','MsgIdFormat',0,'MsgId',1112,'MsgLength',8,'NumSignals',3,'SampleTime',-1,'Signal',struct('SgnName',{'DMC_TempSys','DMC_TempMot','DMC_TempInv'},'SgnStartBit',{24,32,48},'SgnLength',{8,16,16},'SgnType',{0,0,0},'ModeValue',{-1,-1,-1},'DataType',{0,1,1},'ByteLayout',{2,2,2},'Factor',{1,0.5,0.5},'Offset',{-50,0,0},'SgnComment',{{['temperature dmc (inverter)']},{['temperature motor']},{['temperature dmc (inverter)']}},'SgnUnit',{'°C','°C','°C'},'Min',{-50,-16384,-16384},'Max',{205,16383.5,16383.5},'SLDataType',{'SS_DOUBLE','SS_DOUBLE','SS_DOUBLE'}),'MsgIdNumFormat',1,'MsgComment',{{''}}),'Version',1.2,'general',struct('isFromLib',0)),'OFF',[]}},'GroupId',{{struct('Group',{{'RTICAN'}},'No',2,'Behavior',{{'NAMECHANGE'}},'BlockType',{{'SINK'}},'NameChangeFlag',0),'OFF',[]}},'SFcnRTICANMessage',{{struct('MsgType','RX','SFcnPortType','Scalar','MsgName','DMC_TEMP','MsgIdFormat','STD','MsgId',1112,'MsgLength',8,'NumSignals',3,'SampleTime',-1,'Signal',struct('SgnName',{'DMC_TempSys','DMC_TempMot','DMC_TempInv'},'SgnStartBit',{24,32,48},'SgnLength',{8,16,16},'SgnType',{'standard','standard','standard'},'ModeValue',{-1,-1,-1},'DataType',{['unsigned int'],['signed int'],['signed int']},'ByteLayout',{['motorola back.'],['motorola back.'],['motorola back.']},'Factor',{1,0.5,0.5},'Offset',{-50,0,0},'SLDataType',{'SS_DOUBLE','SS_DOUBLE','SS_DOUBLE'}),'StatusSelected','no','TimeSelected','no','DeltaTimeSelected','no','BytePortSelected','no','MessageLengthSelected','no','TriggerPort',struct('Selected','no','TriggerType',0),'UserCoding',struct('Selected','no','InterfaceFile','UserDecodingFile','FcnName','UserDecodeFcn','InportSelected','no','InportWidth',1,'OutportSelected','no','OutportWidth',1),'EnablePortSelected','no','UseRXService','no','BoardType','DS1','BoardNo',1,'ControllerNo',2),'OFF',[]}},'TLCFileName',{{'rtican_rx_message','OFF',[]}})  RTISFcnParameters=struct('SFcnRTICANMessage','struct','TLCFileName','char')  RTIBlockParaDefault=struct('BoardTypeNo',4302,'BoardNo',1,'ChannelNo',1,'Parameters',struct('DataFileSupport',struct('DataFileSelectedMaster',0,'DataFileSelectedLocal',0,'DataFileName','','DataFileDate','','SelectedFile',['<no file selected>']),'Options',struct('StatusSelected',1,'TimeSelected',1,'DeltaTimeSelected',1,'BytePortSelected',0,'MessageLengthSelected',0,'TriggerPort',struct('Selected',0,'TriggerType','rising'),'UserCoding',struct('Selected',0,'InterfaceFile','UserDecodingFile','FcnName','UserDecodeFcn','InportSelected',0,'InportWidth',1,'OutportSelected',0,'OutportWidth',1),'EnablePortSelected',0,'SignalOnPortnameSelected',1,'UseRXService',0),'Message',struct('MsgOnBlocknameSelected',0,'MsgName',['RX Message'],'MsgIdFormat',0,'MsgId',100,'MsgLength',8,'NumSignals',1,'SampleTime',-1,'Signal',struct('SgnName',['RX signal'],'SgnStartBit',0,'SgnLength',8,'SgnType',0,'ModeValue',-1,'DataType',0,'SLDataType','SS_DOUBLE','ByteLayout',0,'Factor',1,'Offset',0,'Min',0,'Max',255,'SgnComment',{{}},'SgnUnit',''),'MsgIdNumFormat',0,'MsgComment',{{''}}),'Version',1.2,'general',struct('isFromLib',1)),'GroupId',struct('Group',{{'RTICAN'}},'No',1,'Behavior',{{'NAMECHANGE'}},'BlockType',{{'SINK'}},'NameChangeFlag',0),'SFcnRTICANMessage',struct('MsgType','RX','MsgName',['RX Message'],'MsgIdFormat','STD','MsgId',100,'MsgLength',8,'NumSignals',1,'SampleTime',-1,'Signal',struct('SgnName',['RX signal'],'SgnStartBit',0,'SgnLength',8,'SgnType','standard','ModeValue',-1,'DataType',['unsigned int'],'ByteLayout',['little endian'],'SLDataType','SS_DOUBLE','Factor',1,'Offset',0),'StatusSelected','yes','TimeSelected','yes','DeltaTimeSelected','yes','BytePortSelected','no','MessageLengthSelected','no','EnablePortSelected','no','UserCoding',struct('Selected','no','InterfaceFile','UserDecodingFile','FcnName','UserDecodeFcn','InportSelected','no','InportWidth',1,'OutportSelected','no','OutportWidth',1),'TriggerPort',struct('Selected','no','TriggerType','rising'),'UseRXService','no','BoardType','DS4302','BoardNo',1,'ControllerNo',1,'SFcnPortType','Scalar'),'TLCFileName','rtican_rx_message')
      settings: AttributesFormatString=Group Id: RTICAN2\n
  DMC_TRQS1 : rtican/RTICAN Receive (RX)   Reserved1=[]  Reserved2=[]  Reserved3=[]  Reserved4=[]  SfcnMessage=[]  Msg_Struct=[]  BoardTypeNo=[]  BoardNo=[]  ChannelNo=[]  Parameters=[]  DialogFcn=[]  UnitName=[]  Revision=[]  UnitValues=[]  DSProperties=struct('RTI',struct('Version',uint32(5),'BlockType',struct('isSLSource',uint8(1),'isSLSink',uint8(1),'isHWSource',uint8(0),'isHWSink',uint8(0),'isSetup',uint8(0),'isInline',uint8(1),'isNonInline',uint8(0),'isInterrupt',uint8(0),'isChannelwise',uint8(0)),'IOBoardType','RTICAN','UnitType','MESSAGE','Identifier','RX','DialogType','MSVC','BlockSet','RTICAN','SlaveProcessor','CAN'))  RTIBlockInterface=struct('OutputPortsWidth',int32([1 1 1 1 1 1 1 1 1 1 1 1 1 1 1 1 1 1 1]),'OutputPortsActive',[1 1 1 1 1 1 1 1 1 1 1 1 1 1 1 1 1 1 1],'OutputPortsName',{{'DMC_SpdAct','DMC_TrqAct','DMC_TrqAvl','DMC_ModelLim','DMC_PowLim','DMC_TrqLim','DMC_IacLim','DMC_TempDmcLim','DMC_SpdLim','DMC_VLim','DMC_CLim','DMC_TrqLimitation','DMC_GenErr','DMC_SensorWarning','DMC_SlewrateLim','DMC_TempMotorLim','DMC_Running','DMC_Ready',['RX status']}},'OutputPortsDataType',{{'SS_DOUBLE','SS_DOUBLE','SS_DOUBLE','SS_DOUBLE','SS_DOUBLE','SS_DOUBLE','SS_DOUBLE','SS_DOUBLE','SS_DOUBLE','SS_DOUBLE','SS_DOUBLE','SS_DOUBLE','SS_DOUBLE','SS_DOUBLE','SS_DOUBLE','SS_DOUBLE','SS_DOUBLE','SS_DOUBLE','SS_DOUBLE'}},'OutputPortsLabel',{{'DMC_SpdAct','DMC_TrqAct','DMC_TrqAvl','DMC_ModelLim','DMC_PowLim','DMC_TrqLim','DMC_IacLim','DMC_TempDmcLim','DMC_SpdLim','DMC_VLim','DMC_CLim','DMC_TrqLimitation','DMC_GenErr','DMC_SensorWarning','DMC_SlewrateLim','DMC_TempMotorLim','DMC_Running','DMC_Ready',''}},'OutputPortsLabelMode','ON','InputPortsWidth',int32(0),'InputPortsActive',0,'DialogFcn','rtican_message_interface_gui','BlockDisplay',{{'','center'}},'IconTransparency','on','ParameterTunableNames',{{}},'InitLevel',3,'BlockName',struct('Token',{{'DMC_TRQS'}}),'SampleTime',{{-1}},'TriggerPort',{{'none'}},'EnablePort',{{'none'}})  RTIBlockParameters=struct('BoardTypeNo',{{1,'OFF',[]}},'BoardNo',{{1,'ON',[1 16]}},'ChannelNo',{{2,'ON',[1 2]}},'Parameters',{{struct('DataFileSupport',struct('DataFileSelectedMaster',1,'DataFileSelectedLocal',1,'DataFileName','c:\users\powertrain_software\desktop\brusa_02-01-02_rev02-2\documentation\dmc5_can_spec_3.9.dbc|','DataFileDate',{{{['14-dec-2011 16:00:26']}}},'SelectedFile','..\brusa_02-01-02_rev02-2\documentation\dmc5_can_spec_3.9.dbc'),'Options',struct('StatusSelected',1,'TimeSelected',0,'DeltaTimeSelected',0,'BytePortSelected',0,'MessageLengthSelected',0,'TriggerPort',struct('Selected',0,'TriggerType',0),'UserCoding',struct('Selected',0,'InterfaceFile','UserDecodingFile','FcnName','UserDecodeFcn','InportSelected',0,'InportWidth',1,'OutportSelected',0,'OutportWidth',1),'EnablePortSelected',0,'SignalOnPortnameSelected',1,'UseRXService',0),'Message',struct('MsgOnBlocknameSelected',1,'MsgName','DMC_TRQS','MsgIdFormat',0,'MsgId',600,'MsgLength',8,'NumSignals',18,'SampleTime',-1,'Signal',struct('SgnName',{'DMC_SpdAct','DMC_TrqAct','DMC_TrqAvl','DMC_ModelLim','DMC_PowLim','DMC_TrqLim','DMC_IacLim','DMC_TempDmcLim','DMC_SpdLim','DMC_VLim','DMC_CLim','DMC_TrqLimitation','DMC_GenErr','DMC_SensorWarning','DMC_SlewrateLim','DMC_TempMotorLim','DMC_Running','DMC_Ready'},'SgnStartBit',{0,16,32,48,49,50,51,52,53,54,55,56,57,58,60,61,62,63},'SgnLength',{16,16,16,1,1,1,1,1,1,1,1,1,1,1,1,1,1,1},'SgnType',{0,0,0,0,0,0,0,0,0,0,0,0,0,0,0,0,0,0},'ModeValue',{-1,-1,-1,-1,-1,-1,-1,-1,-1,-1,-1,-1,-1,-1,-1,-1,-1,-1},'DataType',{1,1,1,0,0,0,0,0,0,0,0,0,0,0,0,0,0,0},'ByteLayout',{2,2,2,2,2,2,2,2,2,2,2,2,2,2,2,2,2,2},'Factor',{1,0.01,0.01,1,1,1,1,1,1,1,1,1,1,1,1,1,1,1},'Offset',{0,0,0,0,0,0,0,0,0,0,0,0,0,0,0,0,0,0},'SgnComment',{{['actual motor speed']},{['actual torque']},{['max available torque']},{['torque limit by motor model']},{['torque limitation by mechanical power']},{['torque limitation by max torque']},{['torque limit by ac current']},{['torque limit by dmc temperature']},{['torque limitation by speed']},{['torque limitation by dc voltage']},{['trq limited by dc current']},{['torque limitation is active']},{['an error bit is set in the error bitmap (DMC_ERR msg)']},{['a warning is set in the warning bitmap (DMC_ERR msg)']},{['torque limitation by max slewrate (torque or speed)']},{['torque limitation by motor temperature']},{['dmc is running']},{['dmc is ready for operation']}},'SgnUnit',{'rpm','Nm','Nm','','','','','','','','','','','','','','',''},'Min',{-32768,-327.68,-327.68,0,0,0,0,0,0,0,0,0,0,0,0,0,0,0},'Max',{23767,327.67,327.67,0,0,0,0,0,0,0,0,0,0,0,0,0,0,0},'SLDataType',{'SS_DOUBLE','SS_DOUBLE','SS_DOUBLE','SS_DOUBLE','SS_DOUBLE','SS_DOUBLE','SS_DOUBLE','SS_DOUBLE','SS_DOUBLE','SS_DOUBLE','SS_DOUBLE','SS_DOUBLE','SS_DOUBLE','SS_DOUBLE','SS_DOUBLE','SS_DOUBLE','SS_DOUBLE','SS_DOUBLE'}),'MsgIdNumFormat',0,'MsgComment',{{''}}),'Version',1.2,'general',struct('isFromLib',0)),'OFF',[]}},'GroupId',{{struct('Group',{{'RTICAN'}},'No',2,'Behavior',{{'NAMECHANGE'}},'BlockType',{{'SINK'}},'NameChangeFlag',0),'OFF',[]}},'SFcnRTICANMessage',{{struct('MsgType','RX','SFcnPortType','Scalar','MsgName','DMC_TRQS','MsgIdFormat','STD','MsgId',600,'MsgLength',8,'NumSignals',18,'SampleTime',-1,'Signal',struct('SgnName',{'DMC_SpdAct','DMC_TrqAct','DMC_TrqAvl','DMC_ModelLim','DMC_PowLim','DMC_TrqLim','DMC_IacLim','DMC_TempDmcLim','DMC_SpdLim','DMC_VLim','DMC_CLim','DMC_TrqLimitation','DMC_GenErr','DMC_SensorWarning','DMC_SlewrateLim','DMC_TempMotorLim','DMC_Running','DMC_Ready'},'SgnStartBit',{0,16,32,48,49,50,51,52,53,54,55,56,57,58,60,61,62,63},'SgnLength',{16,16,16,1,1,1,1,1,1,1,1,1,1,1,1,1,1,1},'SgnType',{'standard','standard','standard','standard','standard','standard','standard','standard','standard','standard','standard','standard','standard','standard','standard','standard','standard','standard'},'ModeValue',{-1,-1,-1,-1,-1,-1,-1,-1,-1,-1,-1,-1,-1,-1,-1,-1,-1,-1},'DataType',{['signed int'],['signed int'],['signed int'],['unsigned int'],['unsigned int'],['unsigned int'],['unsigned int'],['unsigned int'],['unsigned int'],['unsigned int'],['unsigned int'],['unsigned int'],['unsigned int'],['unsigned int'],['unsigned int'],['unsigned int'],['unsigned int'],['unsigned int']},'ByteLayout',{['motorola back.'],['motorola back.'],['motorola back.'],['motorola back.'],['motorola back.'],['motorola back.'],['motorola back.'],['motorola back.'],['motorola back.'],['motorola back.'],['motorola back.'],['motorola back.'],['motorola back.'],['motorola back.'],['motorola back.'],['motorola back.'],['motorola back.'],['motorola back.']},'Factor',{1,0.01,0.01,1,1,1,1,1,1,1,1,1,1,1,1,1,1,1},'Offset',{0,0,0,0,0,0,0,0,0,0,0,0,0,0,0,0,0,0},'SLDataType',{'SS_DOUBLE','SS_DOUBLE','SS_DOUBLE','SS_DOUBLE','SS_DOUBLE','SS_DOUBLE','SS_DOUBLE','SS_DOUBLE','SS_DOUBLE','SS_DOUBLE','SS_DOUBLE','SS_DOUBLE','SS_DOUBLE','SS_DOUBLE','SS_DOUBLE','SS_DOUBLE','SS_DOUBLE','SS_DOUBLE'}),'StatusSelected','yes','TimeSelected','no','DeltaTimeSelected','no','BytePortSelected','no','MessageLengthSelected','no','TriggerPort',struct('Selected','no','TriggerType',0),'UserCoding',struct('Selected','no','InterfaceFile','UserDecodingFile','FcnName','UserDecodeFcn','InportSelected','no','InportWidth',1,'OutportSelected','no','OutportWidth',1),'EnablePortSelected','no','UseRXService','no','BoardType','DS1','BoardNo',1,'ControllerNo',2),'OFF',[]}},'TLCFileName',{{'rtican_rx_message','OFF',[]}})  RTISFcnParameters=struct('SFcnRTICANMessage','struct','TLCFileName','char')  RTIBlockParaDefault=struct('BoardTypeNo',4302,'BoardNo',1,'ChannelNo',1,'Parameters',struct('DataFileSupport',struct('DataFileSelectedMaster',0,'DataFileSelectedLocal',0,'DataFileName','','DataFileDate','','SelectedFile',['<no file selected>']),'Options',struct('StatusSelected',1,'TimeSelected',1,'DeltaTimeSelected',1,'BytePortSelected',0,'MessageLengthSelected',0,'TriggerPort',struct('Selected',0,'TriggerType','rising'),'UserCoding',struct('Selected',0,'InterfaceFile','UserDecodingFile','FcnName','UserDecodeFcn','InportSelected',0,'InportWidth',1,'OutportSelected',0,'OutportWidth',1),'EnablePortSelected',0,'SignalOnPortnameSelected',1,'UseRXService',0),'Message',struct('MsgOnBlocknameSelected',0,'MsgName',['RX Message'],'MsgIdFormat',0,'MsgId',100,'MsgLength',8,'NumSignals',1,'SampleTime',-1,'Signal',struct('SgnName',['RX signal'],'SgnStartBit',0,'SgnLength',8,'SgnType',0,'ModeValue',-1,'DataType',0,'SLDataType','SS_DOUBLE','ByteLayout',0,'Factor',1,'Offset',0,'Min',0,'Max',255,'SgnComment',{{}},'SgnUnit',''),'MsgIdNumFormat',0,'MsgComment',{{''}}),'Version',1.2,'general',struct('isFromLib',1)),'GroupId',struct('Group',{{'RTICAN'}},'No',1,'Behavior',{{'NAMECHANGE'}},'BlockType',{{'SINK'}},'NameChangeFlag',0),'SFcnRTICANMessage',struct('MsgType','RX','MsgName',['RX Message'],'MsgIdFormat','STD','MsgId',100,'MsgLength',8,'NumSignals',1,'SampleTime',-1,'Signal',struct('SgnName',['RX signal'],'SgnStartBit',0,'SgnLength',8,'SgnType','standard','ModeValue',-1,'DataType',['unsigned int'],'ByteLayout',['little endian'],'SLDataType','SS_DOUBLE','Factor',1,'Offset',0),'StatusSelected','yes','TimeSelected','yes','DeltaTimeSelected','yes','BytePortSelected','no','MessageLengthSelected','no','EnablePortSelected','no','UserCoding',struct('Selected','no','InterfaceFile','UserDecodingFile','FcnName','UserDecodeFcn','InportSelected','no','InportWidth',1,'OutportSelected','no','OutportWidth',1),'TriggerPort',struct('Selected','no','TriggerType','rising'),'UseRXService','no','BoardType','DS4302','BoardNo',1,'ControllerNo',1,'SFcnPortType','Scalar'),'TLCFileName','rtican_rx_message')
      settings: AttributesFormatString=Group Id: RTICAN2\n
  DMC_TRQS2 : rtican/RTICAN Receive (RX)   Reserved1=[]  Reserved2=[]  Reserved3=[]  Reserved4=[]  SfcnMessage=[]  Msg_Struct=[]  BoardTypeNo=[]  BoardNo=[]  ChannelNo=[]  Parameters=[]  DialogFcn=[]  UnitName=[]  Revision=[]  UnitValues=[]  DSProperties=struct('RTI',struct('Version',uint32(5),'BlockType',struct('isSLSource',uint8(1),'isSLSink',uint8(1),'isHWSource',uint8(0),'isHWSink',uint8(0),'isSetup',uint8(0),'isInline',uint8(1),'isNonInline',uint8(0),'isInterrupt',uint8(0),'isChannelwise',uint8(0)),'IOBoardType','RTICAN','UnitType','MESSAGE','Identifier','RX','DialogType','MSVC','BlockSet','RTICAN','SlaveProcessor','CAN'))  RTIBlockInterface=struct('OutputPortsWidth',int32([1 1 1]),'OutputPortsActive',[1 1 1],'OutputPortsName',{{'DMC_ActiveLimit','DMC_TrqMin','DMC_TrqMax'}},'OutputPortsDataType',{{'SS_DOUBLE','SS_DOUBLE','SS_DOUBLE'}},'OutputPortsLabel',{{'DMC_ActiveLimit','DMC_TrqMin','DMC_TrqMax'}},'OutputPortsLabelMode','ON','InputPortsWidth',int32(0),'InputPortsActive',0,'DialogFcn','rtican_message_interface_gui','BlockDisplay',{{'','center'}},'IconTransparency','on','ParameterTunableNames',{{}},'InitLevel',3,'BlockName',struct('Token',{{'DMC_TRQS2'}}),'SampleTime',{{-1}},'TriggerPort',{{'none'}},'EnablePort',{{'none'}})  RTIBlockParameters=struct('BoardTypeNo',{{1,'OFF',[]}},'BoardNo',{{1,'ON',[1 16]}},'ChannelNo',{{2,'ON',[1 2]}},'Parameters',{{struct('DataFileSupport',struct('DataFileSelectedMaster',1,'DataFileSelectedLocal',1,'DataFileName','c:\users\powertrain_software\desktop\brusa_02-01-02_rev02-2\documentation\dmc5_can_spec_3.9.dbc|','DataFileDate',{{{['14-dec-2011 16:00:26']}}},'SelectedFile','..\brusa_02-01-02_rev02-2\documentation\dmc5_can_spec_3.9.dbc'),'Options',struct('StatusSelected',0,'TimeSelected',0,'DeltaTimeSelected',0,'BytePortSelected',0,'MessageLengthSelected',0,'TriggerPort',struct('Selected',0,'TriggerType',0),'UserCoding',struct('Selected',0,'InterfaceFile','UserDecodingFile','FcnName','UserDecodeFcn','InportSelected',0,'InportWidth',1,'OutportSelected',0,'OutportWidth',1),'EnablePortSelected',0,'SignalOnPortnameSelected',1,'UseRXService',0),'Message',struct('MsgOnBlocknameSelected',1,'MsgName','DMC_TRQS2','MsgIdFormat',0,'MsgId',616,'MsgLength',8,'NumSignals',3,'SampleTime',-1,'Signal',struct('SgnName',{'DMC_ActiveLimit','DMC_TrqMin','DMC_TrqMax'},'SgnStartBit',{24,32,48},'SgnLength',{8,16,16},'SgnType',{0,0,0},'ModeValue',{-1,-1,-1},'DataType',{0,1,1},'ByteLayout',{2,2,2},'Factor',{1,0.01,0.01},'Offset',{0,0,0},'SgnComment',{{['state number of active limiter']},{['min negative available torque']},{['max positive available torque']}},'SgnUnit',{'','Nm','Nm'},'Min',{0,-327.68,-327.68},'Max',{255,327.67,327.67},'SLDataType',{'SS_DOUBLE','SS_DOUBLE','SS_DOUBLE'}),'MsgIdNumFormat',0,'MsgComment',{{''}}),'Version',1.2,'general',struct('isFromLib',0)),'OFF',[]}},'GroupId',{{struct('Group',{{'RTICAN'}},'No',2,'Behavior',{{'NAMECHANGE'}},'BlockType',{{'SINK'}},'NameChangeFlag',0),'OFF',[]}},'SFcnRTICANMessage',{{struct('MsgType','RX','SFcnPortType','Scalar','MsgName','DMC_TRQS2','MsgIdFormat','STD','MsgId',616,'MsgLength',8,'NumSignals',3,'SampleTime',-1,'Signal',struct('SgnName',{'DMC_ActiveLimit','DMC_TrqMin','DMC_TrqMax'},'SgnStartBit',{24,32,48},'SgnLength',{8,16,16},'SgnType',{'standard','standard','standard'},'ModeValue',{-1,-1,-1},'DataType',{['unsigned int'],['signed int'],['signed int']},'ByteLayout',{['motorola back.'],['motorola back.'],['motorola back.']},'Factor',{1,0.01,0.01},'Offset',{0,0,0},'SLDataType',{'SS_DOUBLE','SS_DOUBLE','SS_DOUBLE'}),'StatusSelected','no','TimeSelected','no','DeltaTimeSelected','no','BytePortSelected','no','MessageLengthSelected','no','TriggerPort',struct('Selected','no','TriggerType',0),'UserCoding',struct('Selected','no','InterfaceFile','UserDecodingFile','FcnName','UserDecodeFcn','InportSelected','no','InportWidth',1,'OutportSelected','no','OutportWidth',1),'EnablePortSelected','no','UseRXService','no','BoardType','DS1','BoardNo',1,'ControllerNo',1),'OFF',[]}},'TLCFileName',{{'rtican_rx_message','OFF',[]}})  RTISFcnParameters=struct('SFcnRTICANMessage','struct','TLCFileName','char')  RTIBlockParaDefault=struct('BoardTypeNo',4302,'BoardNo',1,'ChannelNo',1,'Parameters',struct('DataFileSupport',struct('DataFileSelectedMaster',0,'DataFileSelectedLocal',0,'DataFileName','','DataFileDate','','SelectedFile',['<no file selected>']),'Options',struct('StatusSelected',1,'TimeSelected',1,'DeltaTimeSelected',1,'BytePortSelected',0,'MessageLengthSelected',0,'TriggerPort',struct('Selected',0,'TriggerType','rising'),'UserCoding',struct('Selected',0,'InterfaceFile','UserDecodingFile','FcnName','UserDecodeFcn','InportSelected',0,'InportWidth',1,'OutportSelected',0,'OutportWidth',1),'EnablePortSelected',0,'SignalOnPortnameSelected',1,'UseRXService',0),'Message',struct('MsgOnBlocknameSelected',0,'MsgName',['RX Message'],'MsgIdFormat',0,'MsgId',100,'MsgLength',8,'NumSignals',1,'SampleTime',-1,'Signal',struct('SgnName',['RX signal'],'SgnStartBit',0,'SgnLength',8,'SgnType',0,'ModeValue',-1,'DataType',0,'SLDataType','SS_DOUBLE','ByteLayout',0,'Factor',1,'Offset',0,'Min',0,'Max',255,'SgnComment',{{}},'SgnUnit',''),'MsgIdNumFormat',0,'MsgComment',{{''}}),'Version',1.2,'general',struct('isFromLib',1)),'GroupId',struct('Group',{{'RTICAN'}},'No',1,'Behavior',{{'NAMECHANGE'}},'BlockType',{{'SINK'}},'NameChangeFlag',0),'SFcnRTICANMessage',struct('MsgType','RX','MsgName',['RX Message'],'MsgIdFormat','STD','MsgId',100,'MsgLength',8,'NumSignals',1,'SampleTime',-1,'Signal',struct('SgnName',['RX signal'],'SgnStartBit',0,'SgnLength',8,'SgnType','standard','ModeValue',-1,'DataType',['unsigned int'],'ByteLayout',['little endian'],'SLDataType','SS_DOUBLE','Factor',1,'Offset',0),'StatusSelected','yes','TimeSelected','yes','DeltaTimeSelected','yes','BytePortSelected','no','MessageLengthSelected','no','EnablePortSelected','no','UserCoding',struct('Selected','no','InterfaceFile','UserDecodingFile','FcnName','UserDecodeFcn','InportSelected','no','InportWidth',1,'OutportSelected','no','OutportWidth',1),'TriggerPort',struct('Selected','no','TriggerType','rising'),'UseRXService','no','BoardType','DS4302','BoardNo',1,'ControllerNo',1,'SFcnPortType','Scalar'),'TLCFileName','rtican_rx_message')
      settings: AttributesFormatString=Group Id: RTICAN2\n
  DMC1 : Outport
  DMC2 : Outport  Port=2
  DMC1_ERROR : Outport  Port=3
  DMC2_ERR : Outport  Port=4
  wires:
  DMC_TRQS1/3 -> Bus Creator4/3  "DMC_TrqAvl"
  DMC_ERR/28 -> Bus Creator/28  "DMC_E_SkyVlt"
  DMC2_ERR1/37 -> Bus Creator1/37  "DMC_E_DcCurr"
  DMC2_ERR1/8 -> Bus Creator1/8  "DMC_W_HvUndervoltage"
  DMC_TRQS1/5 -> Bus Creator4/5  "DMC_PowLim"
  DMC_TEMP/2 -> Bus Creator4/21  "DMC_TempMot"
  DMC_TRQS1/6 -> Bus Creator4/6  "DMC_TrqLim"
  DMC_TRQS1/18 -> Bus Creator4/18  "DMC_Ready"
  DMC_ERR/30 -> Bus Creator/30  "DMC_E_ShortCircuit"
  DMC2_ERR1/35 -> Bus Creator1/35  "DMC_E_UV"
  DMC2_TRQS/6 -> Bus Creator2/6  "DMC_TrqLim"
  DMC2_TEMP/2 -> Bus Creator2/21  "DMC_TempMot"
  DMC2_ERR1/21 -> Bus Creator1/21  "DMC_E_OS_Trap"
  DMC2_ERR1/12 -> Bus Creator1/12  "DMC_E_DriverSD"
  DMC2_ERR1/19 -> Bus Creator1/19  "DMC_E_IntSupply"
  DMC_TRQS1/9 -> Bus Creator4/9  "DMC_SpdLim"
  DMC2_ACTV/4 -> Bus Creator2/26  "DMC_DcVltAct"
  DMC2_ERR1/38 -> Bus Creator1/38  "DMC_E_Init"
  Bus Creator2/1 -> DMC2/1
  DMC_ERR/29 -> Bus Creator/29  "DMC_E_VltMeas"
  DMC_TRQS2/1 -> Bus Creator4/27  "DMC_ActiveLimit"
  DMC_TRQS2/3 -> Bus Creator4/29  "DMC_TrqMax"
  DMC_ERR/13 -> Bus Creator/13  "DMC_E_PowerMismatch"
  DMC_TRQS1/8 -> Bus Creator4/8  "DMC_TempDmcLim"
  DMC2_ERR1/14 -> Bus Creator1/14  "DMC_E_CanCtrl2MsgLost"
  DMC_TRQS1/19 -> Bus Creator4/19  "DMC_Status"
  DMC2_ACTV/1 -> Bus Creator2/23  "DMC_MechPwr"
  DMC2_TRQS/16 -> Bus Creator2/16  "DMC_TempMotorLim"
  DMC2_ERR1/36 -> Bus Creator1/36  "DMC_E_OV"
  DMC2_TRQS/7 -> Bus Creator2/7  "DMC_IacLim"
  DMC_ERR/8 -> Bus Creator/8  "DMC_W_HvUndervoltage"
  DMC_ERR/20 -> Bus Creator/20  "DMC_E_AC_Overcurr"
  DMC_ERR/5 -> Bus Creator/5  "DMC_W_DriverSD"
  DMC2_ERR1/7 -> Bus Creator1/7  "DMC_W_SpeedSensor"
  DMC_TEMP/1 -> Bus Creator4/20  "DMC_TempSys"
  DMC_TRQS1/15 -> Bus Creator4/15  "DMC_SlewrateLim"
  DMC_TRQS2/2 -> Bus Creator4/28  "DMC_TrqMin"
  DMC_ERR/31 -> Bus Creator/31  "DMC_E_CanCtrlMsgLost"
  DMC2_TEMP/3 -> Bus Creator2/22  "DMC_TempInv"
  DMC_ERR/19 -> Bus Creator/19  "DMC_E_IntSupply"
  DMC_ERR/12 -> Bus Creator/12  "DMC_E_DriverSD"
  DMC2_ERR1/4 -> Bus Creator1/4  "DMC_I_OscLim_Active"
  DMC_ERR/17 -> Bus Creator/17  "DMC_E_KL15Lost"
  DMC2_TRQS/8 -> Bus Creator2/8  "DMC_TempDmcLim"
  DMC2_ERR1/6 -> Bus Creator1/6  "DMC_W_PowerMismatch"
  DMC_TRQS1/14 -> Bus Creator4/14  "DMC_SensorWarning"
  DMC2_TRQS/10 -> Bus Creator2/10  "DMC_VLim"
  DMC2_TRQS/9 -> Bus Creator2/9  "DMC_SpdLim"
  DMC_ERR/36 -> Bus Creator/36  "DMC_E_OV"
  DMC_TRQS1/10 -> Bus Creator4/10  "DMC_VLim"
  DMC_ACTV/3 -> Bus Creator4/25  "DMC_DcCurrAct"
  DMC2_ERR1/11 -> Bus Creator1/11  "DMC_E_AN_IN"
  DMC2_TRQS2/2 -> Bus Creator2/28  "DMC_TrqMin"
  DMC_TRQS1/7 -> Bus Creator4/7  "DMC_IacLim"
  DMC2_ERR1/1 -> Bus Creator1/1  "DMC_I_SystemCheck"
  DMC_ERR/7 -> Bus Creator/7  "DMC_W_SpeedSensor"
  DMC_ERR/37 -> Bus Creator/37  "DMC_E_DcCurr"
  DMC_TRQS1/4 -> Bus Creator4/4  "DMC_ModelLim"
  DMC_TRQS1/12 -> Bus Creator4/12  "DMC_TrqLimitation"
  DMC2_ERR1/3 -> Bus Creator1/3  "DMC_I_ExtAw1"
  DMC2_ERR1/15 -> Bus Creator1/15  "DMC_E_MotEEPROM"
  DMC_ERR/3 -> Bus Creator/3  "DMC_I_ExtAw1"
  DMC2_ERR1/20 -> Bus Creator1/20  "DMC_E_AC_Overcurr"
  Bus Creator/1 -> DMC1_ERROR/1
  DMC_TRQS1/1 -> Bus Creator4/1  "DMC_SpdAct"
  DMC2_ERR1/23 -> Bus Creator1/23  "DMC_E_SpdSensSupply"
  DMC2_ERR1/30 -> Bus Creator1/30  "DMC_E_ShortCircuit"
  DMC2_ERR1/17 -> Bus Creator1/17  "DMC_E_KL15Lost"
  DMC_ERR/24 -> Bus Creator/24  "DMC_E_SpeedSensor"
  DMC_ERR/10 -> Bus Creator/10  "DMC_W_TempSensor"
  DMC2_TEMP/1 -> Bus Creator2/20  "DMC_TempSys"
  DMC2_ERR1/10 -> Bus Creator1/10  "DMC_W_TempSensor"
  DMC2_ERR1/5 -> Bus Creator1/5  "DMC_W_DriverSD"
  DMC_ERR/26 -> Bus Creator/26  "DMC_E_CanCtrlMsgInvalid"
  DMC2_TRQS/19 -> Bus Creator2/19  "DMC_Status"
  DMC_ERR/6 -> Bus Creator/6  "DMC_W_PowerMismatch"
  DMC2_ERR1/9 -> Bus Creator1/9  "DMC_W_ModMaxLim"
  DMC2_ERR1/22 -> Bus Creator1/22  "DMC_CompatibilityWarnings"
  DMC_ERR/16 -> Bus Creator/16  "DMC_E_Storage"
  DMC_ERR/14 -> Bus Creator/14  "DMC_E_CanCtrl2MsgLost"
  DMC_ERR/21 -> Bus Creator/21  "DMC_E_OS_Trap"
  DMC_ERR/15 -> Bus Creator/15  "DMC_E_MotEEPROM"
  DMC2_TRQS/5 -> Bus Creator2/5  "DMC_PowLim"
  DMC_ERR/32 -> Bus Creator/32  "DMC_E_TempDmc"
  DMC_ERR/25 -> Bus Creator/25  "DMC_E_CanLimMsgInvalid"
  DMC2_ERR1/2 -> Bus Creator1/2  "DMC_I_ExtAw2"
  DMC2_TRQS/13 -> Bus Creator2/13  "DMC_GenErr"
  Bus Creator1/1 -> DMC2_ERR/1
  DMC2_ERR1/25 -> Bus Creator1/25  "DMC_E_CanLimMsgInvalid"
  DMC_ERR/9 -> Bus Creator/9  "DMC_W_ModMaxLim"
  DMC_TRQS1/13 -> Bus Creator4/13  "DMC_GenErr"
  DMC_ERR/4 -> Bus Creator/4  "DMC_I_OscLim_Active"
  DMC_ERR/18 -> Bus Creator/18  "DMC_E_CanComStartup"
  DMC2_ERR1/16 -> Bus Creator1/16  "DMC_E_Storage"
  DMC_ERR/33 -> Bus Creator/33  "DMC_E_TempMot"
  DMC_ACTV/4 -> Bus Creator4/26  "DMC_DcVltAct"
  DMC2_TRQS/17 -> Bus Creator2/17  "DMC_Running"
  DMC2_TRQS/3 -> Bus Creator2/3  "DMC_TrqAvl"
  Bus Creator4/1 -> DMC1/1
  DMC_TEMP/3 -> Bus Creator4/22  "DMC_TempInv"
  DMC_TRQS1/11 -> Bus Creator4/11  "DMC_CLim"
  DMC2_ACTV/3 -> Bus Creator2/25  "DMC_DcCurrAct"
  DMC2_TRQS/4 -> Bus Creator2/4  "DMC_ModelLim"
  DMC2_ERR1/32 -> Bus Creator1/32  "DMC_E_TempDmc"
  DMC2_ACTV/2 -> Bus Creator2/24  "DMC_AcCurrAct"
  DMC_ERR/2 -> Bus Creator/2  "DMC_I_ExtAw2"
  DMC_ACTV/1 -> Bus Creator4/23  "DMC_MechPwr"
  DMC_ERR/11 -> Bus Creator/11  "DMC_E_AN_IN"
  DMC2_ERR1/13 -> Bus Creator1/13  "DMC_E_PowerMismatch"
  DMC2_TRQS/11 -> Bus Creator2/11  "DMC_CLim"
  DMC2_ERR1/33 -> Bus Creator1/33  "DMC_E_TempMot"
  DMC2_TRQS/2 -> Bus Creator2/2  "DMC_TrqAct"
  DMC_ERR/1 -> Bus Creator/1  "DMC_I_SystemCheck"
  DMC2_ERR1/18 -> Bus Creator1/18  "DMC_E_CanComStartup"
  DMC2_ERR1/29 -> Bus Creator1/29  "DMC_E_VltMeas"
  DMC_ERR/23 -> Bus Creator/23  "DMC_E_SpdSensSupply"
  DMC2_ERR1/26 -> Bus Creator1/26  "DMC_E_CanCtrlMsgInvalid"
  DMC_ERR/22 -> Bus Creator/22  "DMC_CompatibilityWarnings"
  DMC2_TRQS/15 -> Bus Creator2/15  "DMC_SlewrateLim"
  DMC2_TRQS/14 -> Bus Creator2/14  "DMC_SensorWarning"
  DMC2_TRQS2/1 -> Bus Creator2/27  "DMC_ActiveLimit"
  DMC_TRQS1/17 -> Bus Creator4/17  "DMC_Running"
  DMC2_ERR1/34 -> Bus Creator1/34  "DMC_E_Speed"
  DMC_ACTV/2 -> Bus Creator4/24  "DMC_AcCurrAct"
  DMC_ERR/34 -> Bus Creator/34  "DMC_E_Speed"
  DMC2_TRQS2/3 -> Bus Creator2/29  "DMC_TrqMax"
  DMC2_TRQS/18 -> Bus Creator2/18  "DMC_Ready"
  DMC_ERR/27 -> Bus Creator/27  "DMC_E_CanLimMsgLost"
  DMC2_TRQS/12 -> Bus Creator2/12  "DMC_TrqLimitation"
  DMC_ERR/35 -> Bus Creator/35  "DMC_E_UV"
  DMC2_ERR1/31 -> Bus Creator1/31  "DMC_E_CanCtrlMsgLost"
  DMC_TRQS1/2 -> Bus Creator4/2  "DMC_TrqAct"
  DMC2_TRQS/1 -> Bus Creator2/1  "DMC_SpdAct"
  DMC2_ERR1/24 -> Bus Creator1/24  "DMC_E_SpeedSensor"
  DMC_ERR/38 -> Bus Creator/38  "DMC_E_Init"
  DMC2_ERR1/28 -> Bus Creator1/28  "DMC_E_SkyVlt"
  DMC2_ERR1/27 -> Bus Creator1/27  "DMC_E_CanLimMsgLost"
  DMC_TRQS1/16 -> Bus Creator4/16  "DMC_TempMotorLim"
